simulink model "IEEE39BusSystem"  (R2024b)
settings: Solver=FixedStepDiscrete  StartTime=0.0  StopTime=15  FixedStep=Ts  MaxStep=1e-4  RelTol=1e-3
PreLoadFcn:
  | Ts = 1/60;
  | EnPSS = 1;
undefined symbols (not defined in the file): Gen1, Gen10, Gen2, Gen3, Gen4, Gen5, Gen6, Gen7, Gen8, Gen9, Load12, Load15, Load16, Load18, Load20, Load21, Load23, Load24, Load25, Load26, Load27, Load28, Load29, Load3, Load31, Load39, Load4, Load7, Load8
libraries: ee_lib x197, fl_lib x97, nesl_utility x91, eeGeneralControl x20, eeSmAC1C x10, eeSmPSS1A x10
(part 2 of 6)

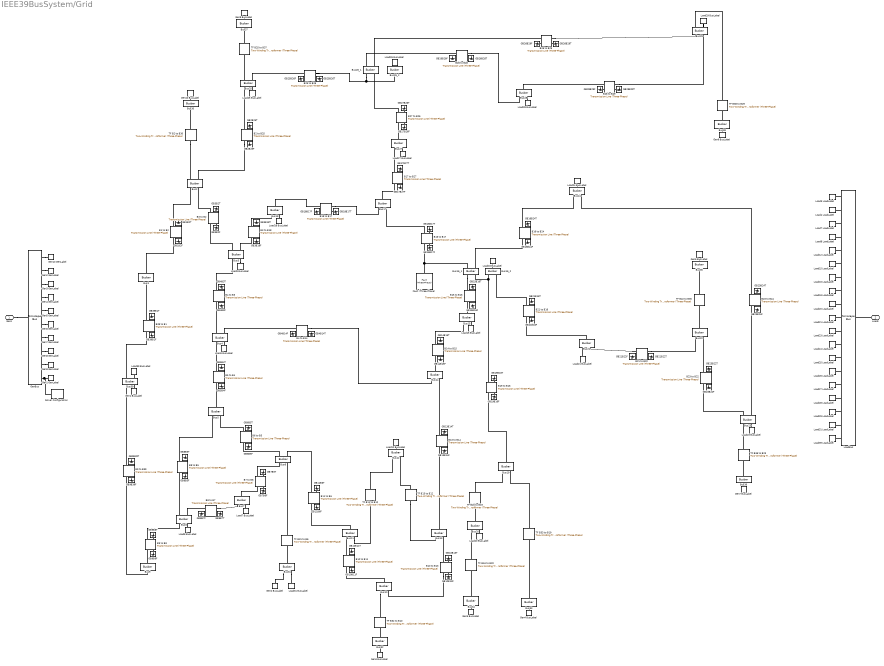
== system IEEE39BusSystem/Grid ==
  B1 to B2 : ee_lib/Passive/Lines/Transmission Line (Three-Phase)  length=1 km  freq=60 Hz  R=16.6635 Ohm/km  L=519.0496 mH/km  M=389.2872 mH/km  Cl=0.20762 uF/km  Cg=0.93427 uF/km  Rm=12.4976 Ohm/km  ModelTwoSections=ee.enum.enable.no  N=1  InterfacePosition=1 km  N1sec=1  N2sec=1  Access_ground=ee.enum.enable.no  R_parasitic=1e-6 Ohm  G_parasitic=1e-6 1/Ohm
      settings: InternalSimscapePortConfiguration="{\"Bottom\":[],\"Left\":[{\"id\":\"N1\",\"label\":\"~1\",\"type\":\"foundation.electrical.three_phase\"},{\"id\":\"g1\",\"label\":\"g1\",\"type\":\"foundation.electrical.electrical\"}],\"Right\":[{\"id\":\"N2\",\"label\":\"~2\",\"type\":\"foundation.electrical.three_phase\"},{\"id\":\"g2\",\"label\":\"g2\",\"type\":\"foundation.electrical.electrical\"}],\"Top\":[]}"
  B10 to B11 : ee_lib/Passive/Lines/Transmission Line (Three-Phase)  length=1 km  freq=60 Hz  R=1.9044 Ohm/km  L=54.3045 mH/km  M=40.7283 mH/km  Cl=0.021662 uF/km  Cg=0.097479 uF/km  Rm=1.4283 Ohm/km  ModelTwoSections=ee.enum.enable.no  N=1  InterfacePosition=1 km  N1sec=1  N2sec=1  Access_ground=ee.enum.enable.no  R_parasitic=1e-6 Ohm  G_parasitic=1e-6 1/Ohm
      settings: InternalSimscapePortConfiguration="{\"Bottom\":[],\"Left\":[{\"id\":\"N1\",\"label\":\"~1\",\"type\":\"foundation.electrical.three_phase\"},{\"id\":\"g1\",\"label\":\"g1\",\"type\":\"foundation.electrical.electrical\"}],\"Right\":[{\"id\":\"N2\",\"label\":\"~2\",\"type\":\"foundation.electrical.three_phase\"},{\"id\":\"g2\",\"label\":\"g2\",\"type\":\"foundation.electrical.electrical\"}],\"Top\":[]}"
  B10 to B13 : ee_lib/Passive/Lines/Transmission Line (Three-Phase)  length=1 km  freq=60 Hz  R=1.9044 Ohm/km  L=54.3045 mH/km  M=40.7283 mH/km  Cl=0.021662 uF/km  Cg=0.097479 uF/km  Rm=1.4283 Ohm/km  ModelTwoSections=ee.enum.enable.no  N=1  InterfacePosition=1 km  N1sec=1  N2sec=1  Access_ground=ee.enum.enable.no  R_parasitic=1e-6 Ohm  G_parasitic=1e-6 1/Ohm
      settings: InternalSimscapePortConfiguration="{\"Bottom\":[],\"Left\":[{\"id\":\"N1\",\"label\":\"~1\",\"type\":\"foundation.electrical.three_phase\"},{\"id\":\"g1\",\"label\":\"g1\",\"type\":\"foundation.electrical.electrical\"}],\"Right\":[{\"id\":\"N2\",\"label\":\"~2\",\"type\":\"foundation.electrical.three_phase\"},{\"id\":\"g2\",\"label\":\"g2\",\"type\":\"foundation.electrical.electrical\"}],\"Top\":[]}"
  B11 to B6 : ee_lib/Passive/Lines/Transmission Line (Three-Phase)  length=1 km  freq=60 Hz  R=3.3327 Ohm/km  L=103.5573 mH/km  M=77.668 mH/km  Cl=0.041274 uF/km  Cg=0.18573 uF/km  Rm=2.4995 Ohm/km  ModelTwoSections=ee.enum.enable.no  N=1  InterfacePosition=1 km  N1sec=1  N2sec=1  Access_ground=ee.enum.enable.no  R_parasitic=1e-6 Ohm  G_parasitic=1e-6 1/Ohm
      settings: InternalSimscapePortConfiguration="{\"Bottom\":[],\"Left\":[{\"id\":\"N1\",\"label\":\"~1\",\"type\":\"foundation.electrical.three_phase\"},{\"id\":\"g1\",\"label\":\"g1\",\"type\":\"foundation.electrical.electrical\"}],\"Right\":[{\"id\":\"N2\",\"label\":\"~2\",\"type\":\"foundation.electrical.three_phase\"},{\"id\":\"g2\",\"label\":\"g2\",\"type\":\"foundation.electrical.electrical\"}],\"Top\":[]}"
  B13 to B14 : ee_lib/Passive/Lines/Transmission Line (Three-Phase)  length=1 km  freq=60 Hz  R=4.2849 Ohm/km  L=127.5523 mH/km  M=95.6643 mH/km  Cl=0.051198 uF/km  Cg=0.23039 uF/km  Rm=3.2137 Ohm/km  ModelTwoSections=ee.enum.enable.no  N=1  InterfacePosition=1 km  N1sec=1  N2sec=1  Access_ground=ee.enum.enable.no  R_parasitic=1e-6 Ohm  G_parasitic=1e-6 1/Ohm
      settings: InternalSimscapePortConfiguration="{\"Bottom\":[],\"Left\":[{\"id\":\"N1\",\"label\":\"~1\",\"type\":\"foundation.electrical.three_phase\"},{\"id\":\"g1\",\"label\":\"g1\",\"type\":\"foundation.electrical.electrical\"}],\"Right\":[{\"id\":\"N2\",\"label\":\"~2\",\"type\":\"foundation.electrical.three_phase\"},{\"id\":\"g2\",\"label\":\"g2\",\"type\":\"foundation.electrical.electrical\"}],\"Top\":[]}"
  B14 to B15 : ee_lib/Passive/Lines/Transmission Line (Three-Phase)  length=1 km  freq=60 Hz  R=8.5698 Ohm/km  L=274.0481 mH/km  M=205.5361 mH/km  Cl=0.10876 uF/km  Cg=0.4894 uF/km  Rm=6.4273 Ohm/km  ModelTwoSections=ee.enum.enable.no  N=1  InterfacePosition=1 km  N1sec=1  N2sec=1  Access_ground=ee.enum.enable.no  R_parasitic=1e-6 Ohm  G_parasitic=1e-6 1/Ohm
      settings: InternalSimscapePortConfiguration="{\"Bottom\":[],\"Left\":[{\"id\":\"N1\",\"label\":\"~1\",\"type\":\"foundation.electrical.three_phase\"},{\"id\":\"g1\",\"label\":\"g1\",\"type\":\"foundation.electrical.electrical\"}],\"Right\":[{\"id\":\"N2\",\"label\":\"~2\",\"type\":\"foundation.electrical.three_phase\"},{\"id\":\"g2\",\"label\":\"g2\",\"type\":\"foundation.electrical.electrical\"}],\"Top\":[]}"
  B15 to B16 : ee_lib/Passive/Lines/Transmission Line (Three-Phase)  length=1 km  freq=60 Hz  R=4.2849 Ohm/km  L=118.7121 mH/km  M=89.0341 mH/km  Cl=0.050812 uF/km  Cg=0.22865 uF/km  Rm=3.2137 Ohm/km  ModelTwoSections=ee.enum.enable.no  N=1  InterfacePosition=1 km  N1sec=1  N2sec=1  Access_ground=ee.enum.enable.no  R_parasitic=1e-6 Ohm  G_parasitic=1e-6 1/Ohm
      settings: InternalSimscapePortConfiguration="{\"Bottom\":[],\"Left\":[{\"id\":\"N1\",\"label\":\"~1\",\"type\":\"foundation.electrical.three_phase\"},{\"id\":\"g1\",\"label\":\"g1\",\"type\":\"foundation.electrical.electrical\"}],\"Right\":[{\"id\":\"N2\",\"label\":\"~2\",\"type\":\"foundation.electrical.three_phase\"},{\"id\":\"g2\",\"label\":\"g2\",\"type\":\"foundation.electrical.electrical\"}],\"Top\":[]}"
  B16 to B17 : ee_lib/Passive/Lines/Transmission Line (Three-Phase)  length=1 km  freq=60 Hz  R=3.3327 Ohm/km  L=112.3976 mH/km  M=84.2982 mH/km  Cl=0.039877 uF/km  Cg=0.17945 uF/km  Rm=2.4995 Ohm/km  ModelTwoSections=ee.enum.enable.no  N=1  InterfacePosition=1 km  N1sec=1  N2sec=1  Access_ground=ee.enum.enable.no  R_parasitic=1e-6 Ohm  G_parasitic=1e-6 1/Ohm
      settings: InternalSimscapePortConfiguration="{\"Bottom\":[],\"Left\":[{\"id\":\"N1\",\"label\":\"~1\",\"type\":\"foundation.electrical.three_phase\"},{\"id\":\"g1\",\"label\":\"g1\",\"type\":\"foundation.electrical.electrical\"}],\"Right\":[{\"id\":\"N2\",\"label\":\"~2\",\"type\":\"foundation.electrical.three_phase\"},{\"id\":\"g2\",\"label\":\"g2\",\"type\":\"foundation.electrical.electrical\"}],\"Top\":[]}"
  B16 to B24 : ee_lib/Passive/Lines/Transmission Line (Three-Phase)  length=1 km  freq=60 Hz  R=1.4283 Ohm/km  L=74.5108 mH/km  M=55.8831 mH/km  Cl=0.020206 uF/km  Cg=0.090927 uF/km  Rm=1.0712 Ohm/km  ModelTwoSections=ee.enum.enable.no  N=1  InterfacePosition=1 km  N1sec=1  N2sec=1  Access_ground=ee.enum.enable.no  R_parasitic=1e-6 Ohm  G_parasitic=1e-6 1/Ohm
      settings: InternalSimscapePortConfiguration="{\"Bottom\":[],\"Left\":[{\"id\":\"N1\",\"label\":\"~1\",\"type\":\"foundation.electrical.three_phase\"},{\"id\":\"g1\",\"label\":\"g1\",\"type\":\"foundation.electrical.electrical\"}],\"Right\":[{\"id\":\"N2\",\"label\":\"~2\",\"type\":\"foundation.electrical.three_phase\"},{\"id\":\"g2\",\"label\":\"g2\",\"type\":\"foundation.electrical.electrical\"}],\"Top\":[]}"
  B17 to B27 : ee_lib/Passive/Lines/Transmission Line (Three-Phase)  length=1 km  freq=60 Hz  R=6.1893 Ohm/km  L=218.4807 mH/km  M=163.8606 mH/km  Cl=0.095562 uF/km  Cg=0.43003 uF/km  Rm=4.642 Ohm/km  ModelTwoSections=ee.enum.enable.no  N=1  InterfacePosition=1 km  N1sec=1  N2sec=1  Access_ground=ee.enum.enable.no  R_parasitic=1e-6 Ohm  G_parasitic=1e-6 1/Ohm
      settings: InternalSimscapePortConfiguration="{\"Bottom\":[],\"Left\":[{\"id\":\"N1\",\"label\":\"~1\",\"type\":\"foundation.electrical.three_phase\"},{\"id\":\"g1\",\"label\":\"g1\",\"type\":\"foundation.electrical.electrical\"}],\"Right\":[{\"id\":\"N2\",\"label\":\"~2\",\"type\":\"foundation.electrical.three_phase\"},{\"id\":\"g2\",\"label\":\"g2\",\"type\":\"foundation.electrical.electrical\"}],\"Top\":[]}"
  B18 to B17 : ee_lib/Passive/Lines/Transmission Line (Three-Phase)  length=1 km  freq=60 Hz  R=3.3327 Ohm/km  L=103.5573 mH/km  M=77.668 mH/km  Cl=0.039194 uF/km  Cg=0.17637 uF/km  Rm=2.4995 Ohm/km  ModelTwoSections=ee.enum.enable.no  N=1  InterfacePosition=1 km  N1sec=1  N2sec=1  Access_ground=ee.enum.enable.no  R_parasitic=1e-6 Ohm  G_parasitic=1e-6 1/Ohm
      settings: InternalSimscapePortConfiguration="{\"Bottom\":[],\"Left\":[{\"id\":\"N1\",\"label\":\"~1\",\"type\":\"foundation.electrical.three_phase\"},{\"id\":\"g1\",\"label\":\"g1\",\"type\":\"foundation.electrical.electrical\"}],\"Right\":[{\"id\":\"N2\",\"label\":\"~2\",\"type\":\"foundation.electrical.three_phase\"},{\"id\":\"g2\",\"label\":\"g2\",\"type\":\"foundation.electrical.electrical\"}],\"Top\":[]}"
  B19 to B16 : ee_lib/Passive/Lines/Transmission Line (Three-Phase)  length=1 km  freq=60 Hz  R=7.6176 Ohm/km  L=246.2644 mH/km  M=184.6983 mH/km  Cl=0.090332 uF/km  Cg=0.4065 uF/km  Rm=5.7132 Ohm/km  ModelTwoSections=ee.enum.enable.no  N=1  InterfacePosition=1 km  N1sec=1  N2sec=1  Access_ground=ee.enum.enable.no  R_parasitic=1e-6 Ohm  G_parasitic=1e-6 1/Ohm
      settings: InternalSimscapePortConfiguration="{\"Bottom\":[],\"Left\":[{\"id\":\"N1\",\"label\":\"~1\",\"type\":\"foundation.electrical.three_phase\"},{\"id\":\"g1\",\"label\":\"g1\",\"type\":\"foundation.electrical.electrical\"}],\"Right\":[{\"id\":\"N2\",\"label\":\"~2\",\"type\":\"foundation.electrical.three_phase\"},{\"id\":\"g2\",\"label\":\"g2\",\"type\":\"foundation.electrical.electrical\"}],\"Top\":[]}"
  B2 to B25 : ee_lib/Passive/Lines/Transmission Line (Three-Phase)  length=1 km  freq=60 Hz  R=33.327 Ohm/km  L=108.6089 mH/km  M=81.4567 mH/km  Cl=0.043383 uF/km  Cg=0.19522 uF/km  Rm=24.9952 Ohm/km  ModelTwoSections=ee.enum.enable.no  N=1  InterfacePosition=1 km  N1sec=1  N2sec=1  Access_ground=ee.enum.enable.no  R_parasitic=1e-6 Ohm  G_parasitic=1e-6 1/Ohm
      settings: InternalSimscapePortConfiguration="{\"Bottom\":[],\"Left\":[{\"id\":\"N1\",\"label\":\"~1\",\"type\":\"foundation.electrical.three_phase\"},{\"id\":\"g1\",\"label\":\"g1\",\"type\":\"foundation.electrical.electrical\"}],\"Right\":[{\"id\":\"N2\",\"label\":\"~2\",\"type\":\"foundation.electrical.three_phase\"},{\"id\":\"g2\",\"label\":\"g2\",\"type\":\"foundation.electrical.electrical\"}],\"Top\":[]}"
  B21 to B16 : ee_lib/Passive/Lines/Transmission Line (Three-Phase)  length=1 km  freq=60 Hz  R=3.8088 Ohm/km  L=170.4908 mH/km  M=127.8681 mH/km  Cl=0.075713 uF/km  Cg=0.34071 uF/km  Rm=2.8566 Ohm/km  ModelTwoSections=ee.enum.enable.no  N=1  InterfacePosition=1 km  N1sec=1  N2sec=1  Access_ground=ee.enum.enable.no  R_parasitic=1e-6 Ohm  G_parasitic=1e-6 1/Ohm
      settings: InternalSimscapePortConfiguration="{\"Bottom\":[],\"Left\":[{\"id\":\"N1\",\"label\":\"~1\",\"type\":\"foundation.electrical.three_phase\"},{\"id\":\"g1\",\"label\":\"g1\",\"type\":\"foundation.electrical.electrical\"}],\"Right\":[{\"id\":\"N2\",\"label\":\"~2\",\"type\":\"foundation.electrical.three_phase\"},{\"id\":\"g2\",\"label\":\"g2\",\"type\":\"foundation.electrical.electrical\"}],\"Top\":[]}"
  B21 to B22 : ee_lib/Passive/Lines/Transmission Line (Three-Phase)  length=1 km  freq=60 Hz  R=3.8088 Ohm/km  L=176.8052 mH/km  M=132.6039 mH/km  Cl=0.076218 uF/km  Cg=0.34298 uF/km  Rm=2.8566 Ohm/km  ModelTwoSections=ee.enum.enable.no  N=1  InterfacePosition=1 km  N1sec=1  N2sec=1  Access_ground=ee.enum.enable.no  R_parasitic=1e-6 Ohm  G_parasitic=1e-6 1/Ohm
      settings: InternalSimscapePortConfiguration="{\"Bottom\":[],\"Left\":[{\"id\":\"N1\",\"label\":\"~1\",\"type\":\"foundation.electrical.three_phase\"},{\"id\":\"g1\",\"label\":\"g1\",\"type\":\"foundation.electrical.electrical\"}],\"Right\":[{\"id\":\"N2\",\"label\":\"~2\",\"type\":\"foundation.electrical.three_phase\"},{\"id\":\"g2\",\"label\":\"g2\",\"type\":\"foundation.electrical.electrical\"}],\"Top\":[]}"
  B23 to B22 : ee_lib/Passive/Lines/Transmission Line (Three-Phase)  length=1 km  freq=60 Hz  R=2.8566 Ohm/km  L=121.2379 mH/km  M=90.9284 mH/km  Cl=0.054853 uF/km  Cg=0.24684 uF/km  Rm=2.1424 Ohm/km  ModelTwoSections=ee.enum.enable.no  N=1  InterfacePosition=1 km  N1sec=1  N2sec=1  Access_ground=ee.enum.enable.no  R_parasitic=1e-6 Ohm  G_parasitic=1e-6 1/Ohm
      settings: InternalSimscapePortConfiguration="{\"Bottom\":[],\"Left\":[{\"id\":\"N1\",\"label\":\"~1\",\"type\":\"foundation.electrical.three_phase\"},{\"id\":\"g1\",\"label\":\"g1\",\"type\":\"foundation.electrical.electrical\"}],\"Right\":[{\"id\":\"N2\",\"label\":\"~2\",\"type\":\"foundation.electrical.three_phase\"},{\"id\":\"g2\",\"label\":\"g2\",\"type\":\"foundation.electrical.electrical\"}],\"Top\":[]}"
  B23 to B24 : ee_lib/Passive/Lines/Transmission Line (Three-Phase)  length=1 km  freq=60 Hz  R=10.4742 Ohm/km  L=442.0131 mH/km  M=331.5098 mH/km  Cl=0.10727 uF/km  Cg=0.48271 uF/km  Rm=7.8557 Ohm/km  ModelTwoSections=ee.enum.enable.no  N=1  InterfacePosition=1 km  N1sec=1  N2sec=1  Access_ground=ee.enum.enable.no  R_parasitic=1e-6 Ohm  G_parasitic=1e-6 1/Ohm
      settings: InternalSimscapePortConfiguration="{\"Bottom\":[],\"Left\":[{\"id\":\"N1\",\"label\":\"~1\",\"type\":\"foundation.electrical.three_phase\"},{\"id\":\"g1\",\"label\":\"g1\",\"type\":\"foundation.electrical.electrical\"}],\"Right\":[{\"id\":\"N2\",\"label\":\"~2\",\"type\":\"foundation.electrical.three_phase\"},{\"id\":\"g2\",\"label\":\"g2\",\"type\":\"foundation.electrical.electrical\"}],\"Top\":[]}"
  B25 to B26 : ee_lib/Passive/Lines/Transmission Line (Three-Phase)  length=1 km  freq=60 Hz  R=15.2352 Ohm/km  L=407.9149 mH/km  M=305.9362 mH/km  Cl=0.15244 uF/km  Cg=0.68596 uF/km  Rm=11.4264 Ohm/km  ModelTwoSections=ee.enum.enable.no  N=1  InterfacePosition=1 km  N1sec=1  N2sec=1  Access_ground=ee.enum.enable.no  R_parasitic=1e-6 Ohm  G_parasitic=1e-6 1/Ohm
      settings: InternalSimscapePortConfiguration="{\"Bottom\":[],\"Left\":[{\"id\":\"N1\",\"label\":\"~1\",\"type\":\"foundation.electrical.three_phase\"},{\"id\":\"g1\",\"label\":\"g1\",\"type\":\"foundation.electrical.electrical\"}],\"Right\":[{\"id\":\"N2\",\"label\":\"~2\",\"type\":\"foundation.electrical.three_phase\"},{\"id\":\"g2\",\"label\":\"g2\",\"type\":\"foundation.electrical.electrical\"}],\"Top\":[]}"
  B26 to B28 : ee_lib/Passive/Lines/Transmission Line (Three-Phase)  length=1 km  freq=60 Hz  R=20.4723 Ohm/km  L=598.612 mH/km  M=448.959 mH/km  Cl=0.23183 uF/km  Cg=1.0432 uF/km  Rm=15.3542 Ohm/km  ModelTwoSections=ee.enum.enable.no  N=1  InterfacePosition=1 km  N1sec=1  N2sec=1  Access_ground=ee.enum.enable.no  R_parasitic=1e-6 Ohm  G_parasitic=1e-6 1/Ohm
      settings: InternalSimscapePortConfiguration="{\"Bottom\":[],\"Left\":[{\"id\":\"N1\",\"label\":\"~1\",\"type\":\"foundation.electrical.three_phase\"},{\"id\":\"g1\",\"label\":\"g1\",\"type\":\"foundation.electrical.electrical\"}],\"Right\":[{\"id\":\"N2\",\"label\":\"~2\",\"type\":\"foundation.electrical.three_phase\"},{\"id\":\"g2\",\"label\":\"g2\",\"type\":\"foundation.electrical.electrical\"}],\"Top\":[]}"
  B26 to B29 : ee_lib/Passive/Lines/Transmission Line (Three-Phase)  length=1 km  freq=60 Hz  R=27.1377 Ohm/km  L=789.309 mH/km  M=591.9818 mH/km  Cl=0.30576 uF/km  Cg=1.3759 uF/km  Rm=20.3533 Ohm/km  ModelTwoSections=ee.enum.enable.no  N=1  InterfacePosition=1 km  N1sec=1  N2sec=1  Access_ground=ee.enum.enable.no  R_parasitic=1e-6 Ohm  G_parasitic=1e-6 1/Ohm
      settings: InternalSimscapePortConfiguration="{\"Bottom\":[],\"Left\":[{\"id\":\"N1\",\"label\":\"~1\",\"type\":\"foundation.electrical.three_phase\"},{\"id\":\"g1\",\"label\":\"g1\",\"type\":\"foundation.electrical.electrical\"}],\"Right\":[{\"id\":\"N2\",\"label\":\"~2\",\"type\":\"foundation.electrical.three_phase\"},{\"id\":\"g2\",\"label\":\"g2\",\"type\":\"foundation.electrical.electrical\"}],\"Top\":[]}"
  B27 to B26 : ee_lib/Passive/Lines/Transmission Line (Three-Phase)  length=1 km  freq=60 Hz  R=6.6654 Ohm/km  L=185.6455 mH/km  M=139.2341 mH/km  Cl=0.071196 uF/km  Cg=0.32038 uF/km  Rm=4.999 Ohm/km  ModelTwoSections=ee.enum.enable.no  N=1  InterfacePosition=1 km  N1sec=1  N2sec=1  Access_ground=ee.enum.enable.no  R_parasitic=1e-6 Ohm  G_parasitic=1e-6 1/Ohm
      settings: InternalSimscapePortConfiguration="{\"Bottom\":[],\"Left\":[{\"id\":\"N1\",\"label\":\"~1\",\"type\":\"foundation.electrical.three_phase\"},{\"id\":\"g1\",\"label\":\"g1\",\"type\":\"foundation.electrical.electrical\"}],\"Right\":[{\"id\":\"N2\",\"label\":\"~2\",\"type\":\"foundation.electrical.three_phase\"},{\"id\":\"g2\",\"label\":\"g2\",\"type\":\"foundation.electrical.electrical\"}],\"Top\":[]}"
  B28 to B29 : ee_lib/Passive/Lines/Transmission Line (Three-Phase)  length=1 km  freq=60 Hz  R=6.6654 Ohm/km  L=190.6971 mH/km  M=143.0228 mH/km  Cl=0.073989 uF/km  Cg=0.33295 uF/km  Rm=4.999 Ohm/km  ModelTwoSections=ee.enum.enable.no  N=1  InterfacePosition=1 km  N1sec=1  N2sec=1  Access_ground=ee.enum.enable.no  R_parasitic=1e-6 Ohm  G_parasitic=1e-6 1/Ohm
      settings: InternalSimscapePortConfiguration="{\"Bottom\":[],\"Left\":[{\"id\":\"N1\",\"label\":\"~1\",\"type\":\"foundation.electrical.three_phase\"},{\"id\":\"g1\",\"label\":\"g1\",\"type\":\"foundation.electrical.electrical\"}],\"Right\":[{\"id\":\"N2\",\"label\":\"~2\",\"type\":\"foundation.electrical.three_phase\"},{\"id\":\"g2\",\"label\":\"g2\",\"type\":\"foundation.electrical.electrical\"}],\"Top\":[]}"
  B3 to B18 : ee_lib/Passive/Lines/Transmission Line (Three-Phase)  length=1 km  freq=60 Hz  R=5.2371 Ohm/km  L=167.965 mH/km  M=125.9737 mH/km  Cl=0.06353 uF/km  Cg=0.28588 uF/km  Rm=3.9278 Ohm/km  ModelTwoSections=ee.enum.enable.no  N=1  InterfacePosition=1 km  N1sec=1  N2sec=1  Access_ground=ee.enum.enable.no  R_parasitic=1e-6 Ohm  G_parasitic=1e-6 1/Ohm
      settings: InternalSimscapePortConfiguration="{\"Bottom\":[],\"Left\":[{\"id\":\"N1\",\"label\":\"~1\",\"type\":\"foundation.electrical.three_phase\"},{\"id\":\"g1\",\"label\":\"g1\",\"type\":\"foundation.electrical.electrical\"}],\"Right\":[{\"id\":\"N2\",\"label\":\"~2\",\"type\":\"foundation.electrical.three_phase\"},{\"id\":\"g2\",\"label\":\"g2\",\"type\":\"foundation.electrical.electrical\"}],\"Top\":[]}"
  B3 to B2 : ee_lib/Passive/Lines/Transmission Line (Three-Phase)  length=1 km  freq=60 Hz  R=6.1893 Ohm/km  L=190.6971 mH/km  M=143.0228 mH/km  Cl=0.076426 uF/km  Cg=0.34392 uF/km  Rm=4.642 Ohm/km  ModelTwoSections=ee.enum.enable.no  N=1  InterfacePosition=1 km  N1sec=1  N2sec=1  Access_ground=ee.enum.enable.no  R_parasitic=1e-6 Ohm  G_parasitic=1e-6 1/Ohm
      settings: InternalSimscapePortConfiguration="{\"Bottom\":[],\"Left\":[{\"id\":\"N1\",\"label\":\"~1\",\"type\":\"foundation.electrical.three_phase\"},{\"id\":\"g1\",\"label\":\"g1\",\"type\":\"foundation.electrical.electrical\"}],\"Right\":[{\"id\":\"N2\",\"label\":\"~2\",\"type\":\"foundation.electrical.three_phase\"},{\"id\":\"g2\",\"label\":\"g2\",\"type\":\"foundation.electrical.electrical\"}],\"Top\":[]}"
  B39 to B1 : ee_lib/Passive/Lines/Transmission Line (Three-Phase)  length=1 km  freq=60 Hz  R=4.761 Ohm/km  L=315.7236 mH/km  M=236.7927 mH/km  Cl=0.22286 uF/km  Cg=1.0029 uF/km  Rm=3.5707 Ohm/km  ModelTwoSections=ee.enum.enable.no  N=1  InterfacePosition=1 km  N1sec=1  N2sec=1  Access_ground=ee.enum.enable.no  R_parasitic=1e-6 Ohm  G_parasitic=1e-6 1/Ohm
      settings: InternalSimscapePortConfiguration="{\"Bottom\":[],\"Left\":[{\"id\":\"N1\",\"label\":\"~1\",\"type\":\"foundation.electrical.three_phase\"},{\"id\":\"g1\",\"label\":\"g1\",\"type\":\"foundation.electrical.electrical\"}],\"Right\":[{\"id\":\"N2\",\"label\":\"~2\",\"type\":\"foundation.electrical.three_phase\"},{\"id\":\"g2\",\"label\":\"g2\",\"type\":\"foundation.electrical.electrical\"}],\"Top\":[]}"
  B4 to B14 : ee_lib/Passive/Lines/Transmission Line (Three-Phase)  length=1 km  freq=60 Hz  R=3.8088 Ohm/km  L=162.9134 mH/km  M=122.185 mH/km  Cl=0.041066 uF/km  Cg=0.18479 uF/km  Rm=2.8566 Ohm/km  ModelTwoSections=ee.enum.enable.no  N=1  InterfacePosition=1 km  N1sec=1  N2sec=1  Access_ground=ee.enum.enable.no  R_parasitic=1e-6 Ohm  G_parasitic=1e-6 1/Ohm
      settings: InternalSimscapePortConfiguration="{\"Bottom\":[],\"Left\":[{\"id\":\"N1\",\"label\":\"~1\",\"type\":\"foundation.electrical.three_phase\"},{\"id\":\"g1\",\"label\":\"g1\",\"type\":\"foundation.electrical.electrical\"}],\"Right\":[{\"id\":\"N2\",\"label\":\"~2\",\"type\":\"foundation.electrical.three_phase\"},{\"id\":\"g2\",\"label\":\"g2\",\"type\":\"foundation.electrical.electrical\"}],\"Top\":[]}"
  B4 to B3 : ee_lib/Passive/Lines/Transmission Line (Three-Phase)  length=1 km  freq=60 Hz  R=6.1893 Ohm/km  L=268.9965 mH/km  M=201.7474 mH/km  Cl=0.065788 uF/km  Cg=0.29605 uF/km  Rm=4.642 Ohm/km  ModelTwoSections=ee.enum.enable.no  N=1  InterfacePosition=1 km  N1sec=1  N2sec=1  Access_ground=ee.enum.enable.no  R_parasitic=1e-6 Ohm  G_parasitic=1e-6 1/Ohm
      settings: InternalSimscapePortConfiguration="{\"Bottom\":[],\"Left\":[{\"id\":\"N1\",\"label\":\"~1\",\"type\":\"foundation.electrical.three_phase\"},{\"id\":\"g1\",\"label\":\"g1\",\"type\":\"foundation.electrical.electrical\"}],\"Right\":[{\"id\":\"N2\",\"label\":\"~2\",\"type\":\"foundation.electrical.three_phase\"},{\"id\":\"g2\",\"label\":\"g2\",\"type\":\"foundation.electrical.electrical\"}],\"Top\":[]}"
  B5 to B4 : ee_lib/Passive/Lines/Transmission Line (Three-Phase)  length=1 km  freq=60 Hz  R=3.8088 Ohm/km  L=162.9134 mH/km  M=122.185 mH/km  Cl=0.041066 uF/km  Cg=0.18479 uF/km  Rm=2.8566 Ohm/km  ModelTwoSections=ee.enum.enable.no  N=1  InterfacePosition=1 km  N1sec=1  N2sec=1  Access_ground=ee.enum.enable.no  R_parasitic=1e-6 Ohm  G_parasitic=1e-6 1/Ohm
      settings: InternalSimscapePortConfiguration="{\"Bottom\":[],\"Left\":[{\"id\":\"N1\",\"label\":\"~1\",\"type\":\"foundation.electrical.three_phase\"},{\"id\":\"g1\",\"label\":\"g1\",\"type\":\"foundation.electrical.electrical\"}],\"Right\":[{\"id\":\"N2\",\"label\":\"~2\",\"type\":\"foundation.electrical.three_phase\"},{\"id\":\"g2\",\"label\":\"g2\",\"type\":\"foundation.electrical.electrical\"}],\"Top\":[]}"
  B6 to B5 : ee_lib/Passive/Lines/Transmission Line (Three-Phase)  length=1 km  freq=60 Hz  R=0.9522 Ohm/km  L=32.8353 mH/km  M=24.6264 mH/km  Cl=0.012896 uF/km  Cg=0.058033 uF/km  Rm=0.71415 Ohm/km  ModelTwoSections=ee.enum.enable.no  N=1  InterfacePosition=1 km  N1sec=1  N2sec=1  Access_ground=ee.enum.enable.no  R_parasitic=1e-6 Ohm  G_parasitic=1e-6 1/Ohm
      settings: InternalSimscapePortConfiguration="{\"Bottom\":[],\"Left\":[{\"id\":\"N1\",\"label\":\"~1\",\"type\":\"foundation.electrical.three_phase\"},{\"id\":\"g1\",\"label\":\"g1\",\"type\":\"foundation.electrical.electrical\"}],\"Right\":[{\"id\":\"N2\",\"label\":\"~2\",\"type\":\"foundation.electrical.three_phase\"},{\"id\":\"g2\",\"label\":\"g2\",\"type\":\"foundation.electrical.electrical\"}],\"Top\":[]}"
  B7 to B6 : ee_lib/Passive/Lines/Transmission Line (Three-Phase)  length=1 km  freq=60 Hz  R=2.8566 Ohm/km  L=116.1863 mH/km  M=87.1397 mH/km  Cl=0.033577 uF/km  Cg=0.1511 uF/km  Rm=2.1424 Ohm/km  ModelTwoSections=ee.enum.enable.no  N=1  InterfacePosition=1 km  N1sec=1  N2sec=1  Access_ground=ee.enum.enable.no  R_parasitic=1e-6 Ohm  G_parasitic=1e-6 1/Ohm
      settings: InternalSimscapePortConfiguration="{\"Bottom\":[],\"Left\":[{\"id\":\"N1\",\"label\":\"~1\",\"type\":\"foundation.electrical.three_phase\"},{\"id\":\"g1\",\"label\":\"g1\",\"type\":\"foundation.electrical.electrical\"}],\"Right\":[{\"id\":\"N2\",\"label\":\"~2\",\"type\":\"foundation.electrical.three_phase\"},{\"id\":\"g2\",\"label\":\"g2\",\"type\":\"foundation.electrical.electrical\"}],\"Top\":[]}"
  B8 to B5 : ee_lib/Passive/Lines/Transmission Line (Three-Phase)  length=1 km  freq=60 Hz  R=3.8088 Ohm/km  L=141.4442 mH/km  M=106.0831 mH/km  Cl=0.043859 uF/km  Cg=0.19736 uF/km  Rm=2.8566 Ohm/km  ModelTwoSections=ee.enum.enable.no  N=1  InterfacePosition=1 km  N1sec=1  N2sec=1  Access_ground=ee.enum.enable.no  R_parasitic=1e-6 Ohm  G_parasitic=1e-6 1/Ohm
      settings: InternalSimscapePortConfiguration="{\"Bottom\":[],\"Left\":[{\"id\":\"N1\",\"label\":\"~1\",\"type\":\"foundation.electrical.three_phase\"},{\"id\":\"g1\",\"label\":\"g1\",\"type\":\"foundation.electrical.electrical\"}],\"Right\":[{\"id\":\"N2\",\"label\":\"~2\",\"type\":\"foundation.electrical.three_phase\"},{\"id\":\"g2\",\"label\":\"g2\",\"type\":\"foundation.electrical.electrical\"}],\"Top\":[]}"
  B8 to B7 : ee_lib/Passive/Lines/Transmission Line (Three-Phase)  length=1 km  freq=60 Hz  R=1.9044 Ohm/km  L=58.0931 mH/km  M=43.5699 mH/km  Cl=0.023177 uF/km  Cg=0.1043 uF/km  Rm=1.4283 Ohm/km  ModelTwoSections=ee.enum.enable.no  N=1  InterfacePosition=1 km  N1sec=1  N2sec=1  Access_ground=ee.enum.enable.no  R_parasitic=1e-6 Ohm  G_parasitic=1e-6 1/Ohm
      settings: InternalSimscapePortConfiguration="{\"Bottom\":[],\"Left\":[{\"id\":\"N1\",\"label\":\"~1\",\"type\":\"foundation.electrical.three_phase\"},{\"id\":\"g1\",\"label\":\"g1\",\"type\":\"foundation.electrical.electrical\"}],\"Right\":[{\"id\":\"N2\",\"label\":\"~2\",\"type\":\"foundation.electrical.three_phase\"},{\"id\":\"g2\",\"label\":\"g2\",\"type\":\"foundation.electrical.electrical\"}],\"Top\":[]}"
  B9 to B39 : ee_lib/Passive/Lines/Transmission Line (Three-Phase)  length=1 km  freq=60 Hz  R=4.761 Ohm/km  L=315.7236 mH/km  M=236.7927 mH/km  Cl=0.35657 uF/km  Cg=1.6046 uF/km  Rm=3.5707 Ohm/km  ModelTwoSections=ee.enum.enable.no  N=1  InterfacePosition=1 km  N1sec=1  N2sec=1  Access_ground=ee.enum.enable.no  R_parasitic=1e-6 Ohm  G_parasitic=1e-6 1/Ohm
      settings: InternalSimscapePortConfiguration="{\"Bottom\":[],\"Left\":[{\"id\":\"N1\",\"label\":\"~1\",\"type\":\"foundation.electrical.three_phase\"},{\"id\":\"g1\",\"label\":\"g1\",\"type\":\"foundation.electrical.electrical\"}],\"Right\":[{\"id\":\"N2\",\"label\":\"~2\",\"type\":\"foundation.electrical.three_phase\"},{\"id\":\"g2\",\"label\":\"g2\",\"type\":\"foundation.electrical.electrical\"}],\"Top\":[]}"
  B9 to B8 : ee_lib/Passive/Lines/Transmission Line (Three-Phase)  length=1 km  freq=60 Hz  R=10.9503 Ohm/km  L=458.4307 mH/km  M=343.823 mH/km  Cl=0.11303 uF/km  Cg=0.50865 uF/km  Rm=8.2127 Ohm/km  ModelTwoSections=ee.enum.enable.no  N=1  InterfacePosition=1 km  N1sec=1  N2sec=1  Access_ground=ee.enum.enable.no  R_parasitic=1e-6 Ohm  G_parasitic=1e-6 1/Ohm
      settings: InternalSimscapePortConfiguration="{\"Bottom\":[],\"Left\":[{\"id\":\"N1\",\"label\":\"~1\",\"type\":\"foundation.electrical.three_phase\"},{\"id\":\"g1\",\"label\":\"g1\",\"type\":\"foundation.electrical.electrical\"}],\"Right\":[{\"id\":\"N2\",\"label\":\"~2\",\"type\":\"foundation.electrical.three_phase\"},{\"id\":\"g2\",\"label\":\"g2\",\"type\":\"foundation.electrical.electrical\"}],\"Top\":[]}"
  Bus1 : ee_lib/Connectors & References/Busbar  Tag="1.036 pu\\n20.85 deg\\n-150.3  150.3 MW\\n19.1  -19.1 Mvar"  n_nodes=ee.enum.connectors.busbar_number_of_connections.two  VRated=345 kV  freq=60 Hz  show_ps=ee.enum.connectors.busbar_measurement.false
      settings: AttributesFormatString=%<Tag>  InternalSimscapePortConfiguration="{\"Bottom\":[],\"Left\":[{\"id\":\"N1\",\"label\":\"~1\",\"type\":\"foundation.electrical.three_phase\"}],\"Right\":[{\"id\":\"N2\",\"label\":\"~2\",\"type\":\"foundation.electrical.three_phase\"}],\"Top\":[]}"
  Bus10 : ee_lib/Connectors & References/Busbar  Tag="0.966 pu\\n25.54 deg\\n649.4 -366.4 -283.0 MW\\n36.0  -34.5   -1.5 Mvar"  n_nodes=ee.enum.connectors.busbar_number_of_connections.three  VRated=345 kV  freq=60 Hz  show_ps=ee.enum.connectors.busbar_measurement.false
      settings: AttributesFormatString=%<Tag>  InternalSimscapePortConfiguration="{\"Bottom\":[],\"Left\":[{\"id\":\"N1\",\"label\":\"~1\",\"type\":\"foundation.electrical.three_phase\"},{\"id\":\"N3\",\"label\":\"~3\",\"type\":\"foundation.electrical.three_phase\"}],\"Right\":[{\"id\":\"N2\",\"label\":\"~2\",\"type\":\"foundation.electrical.three_phase\"}],\"Top\":[]}"
  Bus11 : ee_lib/Connectors & References/Busbar  Tag="0.963 pu\\n24.57 deg\\n365.8 -365.8   -0.0 MW\\n35.0    3.5  -38.4 Mvar"  n_nodes=ee.enum.connectors.busbar_number_of_connections.three  VRated=345 kV  freq=60 Hz  show_ps=ee.enum.connectors.busbar_measurement.false
      settings: AttributesFormatString=%<Tag>  InternalSimscapePortConfiguration="{\"Bottom\":[],\"Left\":[{\"id\":\"N1\",\"label\":\"~1\",\"type\":\"foundation.electrical.three_phase\"},{\"id\":\"N3\",\"label\":\"~3\",\"type\":\"foundation.electrical.three_phase\"}],\"Right\":[{\"id\":\"N2\",\"label\":\"~2\",\"type\":\"foundation.electrical.three_phase\"}],\"Top\":[]}"
  Bus12 : ee_lib/Connectors & References/Busbar  Tag="0.945 pu\\n54.61 deg\\n-0.2   -7.6    7.8 MW\\n37.6  -78.6   41.1 Mvar"  n_nodes=ee.enum.connectors.busbar_number_of_connections.three  VRated=345 kV  freq=60 Hz  show_ps=ee.enum.connectors.busbar_measurement.false
      settings: AttributesFormatString=%<Tag>  InternalSimscapePortConfiguration="{\"Bottom\":[],\"Left\":[{\"id\":\"N1\",\"label\":\"~1\",\"type\":\"foundation.electrical.three_phase\"},{\"id\":\"N3\",\"label\":\"~3\",\"type\":\"foundation.electrical.three_phase\"}],\"Right\":[{\"id\":\"N2\",\"label\":\"~2\",\"type\":\"foundation.electrical.three_phase\"}],\"Top\":[]}"
  Bus13 : ee_lib/Connectors & References/Busbar  Tag="0.964 pu\\n24.79 deg\\n-8.0 -274.7  282.6 MW\\n-42.1   37.5    4.6 Mvar"  n_nodes=ee.enum.connectors.busbar_number_of_connections.three  VRated=345 kV  freq=60 Hz  show_ps=ee.enum.connectors.busbar_measurement.false
      settings: AttributesFormatString=%<Tag>  InternalSimscapePortConfiguration="{\"Bottom\":[],\"Left\":[{\"id\":\"N1\",\"label\":\"~1\",\"type\":\"foundation.electrical.three_phase\"},{\"id\":\"N3\",\"label\":\"~3\",\"type\":\"foundation.electrical.three_phase\"}],\"Right\":[{\"id\":\"N2\",\"label\":\"~2\",\"type\":\"foundation.electrical.three_phase\"}],\"Top\":[]}"
  Bus14 : ee_lib/Connectors & References/Busbar  Tag="0.965 pu\\n23.06 deg\\n-267.1   -6.8  273.9 MW\\n-19.3   49.0  -29.7 Mvar"  n_nodes=ee.enum.connectors.busbar_number_of_connections.three  VRated=345 kV  freq=60 Hz  show_ps=ee.enum.connectors.busbar_measurement.false
      settings: AttributesFormatString=%<Tag>  InternalSimscapePortConfiguration="{\"Bottom\":[],\"Left\":[{\"id\":\"N1\",\"label\":\"~1\",\"type\":\"foundation.electrical.three_phase\"},{\"id\":\"N3\",\"label\":\"~3\",\"type\":\"foundation.electrical.three_phase\"}],\"Right\":[{\"id\":\"N2\",\"label\":\"~2\",\"type\":\"foundation.electrical.three_phase\"}],\"Top\":[]}"
  Bus15 : ee_lib/Connectors & References/Busbar  Tag="0.972 pu\\n22.94 deg\\n6.8  295.8 -302.6 MW\\n-14.9  159.6 -144.7 Mvar"  n_nodes=ee.enum.connectors.busbar_number_of_connections.three  VRated=345 kV  freq=60 Hz  show_ps=ee.enum.connectors.busbar_measurement.false
      settings: AttributesFormatString=%<Tag>  InternalSimscapePortConfiguration="{\"Bottom\":[],\"Left\":[{\"id\":\"N1\",\"label\":\"~1\",\"type\":\"foundation.electrical.three_phase\"},{\"id\":\"N3\",\"label\":\"~3\",\"type\":\"foundation.electrical.three_phase\"}],\"Right\":[{\"id\":\"N2\",\"label\":\"~2\",\"type\":\"foundation.electrical.three_phase\"}],\"Top\":[]}"
  Bus16_1 : ee_lib/Connectors & References/Busbar  Tag="0.990 pu\\n24.51 deg\\n-296.9 -261.2  518.6   39.4 MW\\n-154.1   70.5  -52.7  136.3 Mvar"  n_nodes=ee.enum.connectors.busbar_number_of_connections.four  VRated=345 kV  freq=60 Hz  show_ps=ee.enum.connectors.busbar_measurement.false
      settings: AttributesFormatString=%<Tag>  InternalSimscapePortConfiguration="{\"Bottom\":[],\"Left\":[{\"id\":\"N1\",\"label\":\"~1\",\"type\":\"foundation.electrical.three_phase\"},{\"id\":\"N3\",\"label\":\"~3\",\"type\":\"foundation.electrical.three_phase\"}],\"Right\":[{\"id\":\"N2\",\"label\":\"~2\",\"type\":\"foundation.electrical.three_phase\"},{\"id\":\"N4\",\"label\":\"~4\",\"type\":\"foundation.electrical.three_phase\"}],\"Top\":[]}"
  Bus16_2 : ee_lib/Connectors & References/Busbar  Tag="0.990 pu\\n24.51 deg\\n-1.7 -322.6  324.3 MW\\n-0.2  -31.7   31.9 Mvar"  n_nodes=ee.enum.connectors.busbar_number_of_connections.three  VRated=345 kV  freq=60 Hz  show_ps=ee.enum.connectors.busbar_measurement.false
      settings: AttributesFormatString=%<Tag>  InternalSimscapePortConfiguration="{\"Bottom\":[],\"Left\":[{\"id\":\"N1\",\"label\":\"~1\",\"type\":\"foundation.electrical.three_phase\"},{\"id\":\"N3\",\"label\":\"~3\",\"type\":\"foundation.electrical.three_phase\"}],\"Right\":[{\"id\":\"N2\",\"label\":\"~2\",\"type\":\"foundation.electrical.three_phase\"}],\"Top\":[]}"
  Bus17 : ee_lib/Connectors & References/Busbar  Tag="0.994 pu\\n23.13 deg\\n-215.0  -45.6  260.6 MW\\n4.7   59.1  -63.9 Mvar"  n_nodes=ee.enum.connectors.busbar_number_of_connections.three  VRated=345 kV  freq=60 Hz  show_ps=ee.enum.connectors.busbar_measurement.false
      settings: AttributesFormatString=%<Tag>  InternalSimscapePortConfiguration="{\"Bottom\":[],\"Left\":[{\"id\":\"N1\",\"label\":\"~1\",\"type\":\"foundation.electrical.three_phase\"},{\"id\":\"N3\",\"label\":\"~3\",\"type\":\"foundation.electrical.three_phase\"}],\"Right\":[{\"id\":\"N2\",\"label\":\"~2\",\"type\":\"foundation.electrical.three_phase\"}],\"Top\":[]}"
  Bus18 : ee_lib/Connectors & References/Busbar  Tag="0.993 pu\\n22.11 deg\\n-58.9  214.7 -155.8 MW\\n25.1    4.5  -29.6 Mvar"  n_nodes=ee.enum.connectors.busbar_number_of_connections.three  VRated=345 kV  freq=60 Hz  show_ps=ee.enum.connectors.busbar_measurement.false
      settings: AttributesFormatString=%<Tag>  InternalSimscapePortConfiguration="{\"Bottom\":[],\"Left\":[{\"id\":\"N1\",\"label\":\"~1\",\"type\":\"foundation.electrical.three_phase\"},{\"id\":\"N3\",\"label\":\"~3\",\"type\":\"foundation.electrical.three_phase\"}],\"Right\":[{\"id\":\"N2\",\"label\":\"~2\",\"type\":\"foundation.electrical.three_phase\"}],\"Top\":[]}"
  Bus19 : ee_lib/Connectors & References/Busbar  Tag="0.991 pu\\n30.48 deg\\n-107.6 -521.4  629.0 MW\\n-15.6   28.7  -13.2 Mvar"  n_nodes=ee.enum.connectors.busbar_number_of_connections.three  VRated=345 kV  freq=60 Hz  show_ps=ee.enum.connectors.busbar_measurement.false
      settings: AttributesFormatString=%<Tag>  InternalSimscapePortConfiguration="{\"Bottom\":[],\"Left\":[{\"id\":\"N1\",\"label\":\"~1\",\"type\":\"foundation.electrical.three_phase\"},{\"id\":\"N3\",\"label\":\"~3\",\"type\":\"foundation.electrical.three_phase\"}],\"Right\":[{\"id\":\"N2\",\"label\":\"~2\",\"type\":\"foundation.electrical.three_phase\"}],\"Top\":[]}"
  Bus2 : ee_lib/Connectors & References/Busbar  Tag="1.020 pu\\n24.31 deg\\n-151.1  249.7 -325.3  226.7 MW\\n83.1  145.9 -143.0  -86.0 Mvar"  n_nodes=ee.enum.connectors.busbar_number_of_connections.four  VRated=345 kV  freq=60 Hz  show_ps=ee.enum.connectors.busbar_measurement.false
      settings: AttributesFormatString=%<Tag>  InternalSimscapePortConfiguration="{\"Bottom\":[],\"Left\":[{\"id\":\"N1\",\"label\":\"~1\",\"type\":\"foundation.electrical.three_phase\"},{\"id\":\"N3\",\"label\":\"~3\",\"type\":\"foundation.electrical.three_phase\"}],\"Right\":[{\"id\":\"N2\",\"label\":\"~2\",\"type\":\"foundation.electrical.three_phase\"},{\"id\":\"N4\",\"label\":\"~4\",\"type\":\"foundation.electrical.three_phase\"}],\"Top\":[]}"
  Bus20 : ee_lib/Connectors & References/Busbar  Tag="0.988 pu\\n29.61 deg\\n505.4  107.3 -612.7 MW\\n86.8   13.7 -100.5 Mvar"  n_nodes=ee.enum.connectors.busbar_number_of_connections.three  VRated=345 kV  freq=60 Hz  show_ps=ee.enum.connectors.busbar_measurement.false
      settings: AttributesFormatString=%<Tag>  InternalSimscapePortConfiguration="{\"Bottom\":[],\"Left\":[{\"id\":\"N1\",\"label\":\"~1\",\"type\":\"foundation.electrical.three_phase\"},{\"id\":\"N3\",\"label\":\"~3\",\"type\":\"foundation.electrical.three_phase\"}],\"Right\":[{\"id\":\"N2\",\"label\":\"~2\",\"type\":\"foundation.electrical.three_phase\"}],\"Top\":[]}"
  Bus21 : ee_lib/Connectors & References/Busbar  Tag="0.996 pu\\n27.05 deg\\n-272.0 -325.1  597.2 MW\\n-114.2  -21.3  135.5 Mvar"  n_nodes=ee.enum.connectors.busbar_number_of_connections.three  VRated=345 kV  freq=60 Hz  show_ps=ee.enum.connectors.busbar_measurement.false
      settings: AttributesFormatString=%<Tag>  InternalSimscapePortConfiguration="{\"Bottom\":[],\"Left\":[{\"id\":\"N1\",\"label\":\"~1\",\"type\":\"foundation.electrical.three_phase\"},{\"id\":\"N3\",\"label\":\"~3\",\"type\":\"foundation.electrical.three_phase\"}],\"Right\":[{\"id\":\"N2\",\"label\":\"~2\",\"type\":\"foundation.electrical.three_phase\"}],\"Top\":[]}"
  Bus22 : ee_lib/Connectors & References/Busbar  Tag="1.022 pu\\n31.70 deg\\n-600.2  649.4  -49.2 MW\\n-161.8  163.5   -1.8 Mvar"  n_nodes=ee.enum.connectors.busbar_number_of_connections.three  VRated=345 kV  freq=60 Hz  show_ps=ee.enum.connectors.busbar_measurement.false
      settings: AttributesFormatString=%<Tag>  InternalSimscapePortConfiguration="{\"Bottom\":[],\"Left\":[{\"id\":\"N1\",\"label\":\"~1\",\"type\":\"foundation.electrical.three_phase\"},{\"id\":\"N3\",\"label\":\"~3\",\"type\":\"foundation.electrical.three_phase\"}],\"Right\":[{\"id\":\"N2\",\"label\":\"~2\",\"type\":\"foundation.electrical.three_phase\"}],\"Top\":[]}"
  Bus23 : ee_lib/Connectors & References/Busbar  Tag="1.020 pu\\n31.45 deg\\n558.2   49.2 -257.7 -349.7 MW\\n112.0   20.8  -88.1  -44.7 Mvar"  n_nodes=ee.enum.connectors.busbar_number_of_connections.four  VRated=345 kV  freq=60 Hz  show_ps=ee.enum.connectors.busbar_measurement.false
      settings: AttributesFormatString=%<Tag>  InternalSimscapePortConfiguration="{\"Bottom\":[],\"Left\":[{\"id\":\"N1\",\"label\":\"~1\",\"type\":\"foundation.electrical.three_phase\"},{\"id\":\"N3\",\"label\":\"~3\",\"type\":\"foundation.electrical.three_phase\"}],\"Right\":[{\"id\":\"N2\",\"label\":\"~2\",\"type\":\"foundation.electrical.three_phase\"},{\"id\":\"N4\",\"label\":\"~4\",\"type\":\"foundation.electrical.three_phase\"}],\"Top\":[]}"
  Bus24 : ee_lib/Connectors & References/Busbar  Tag="0.998 pu\\n24.62 deg\\n-39.5 -307.5  347.0 MW\\n-130.7   91.7   39.1 Mvar"  n_nodes=ee.enum.connectors.busbar_number_of_connections.three  VRated=345 kV  freq=60 Hz  show_ps=ee.enum.connectors.busbar_measurement.false
      settings: AttributesFormatString=%<Tag>  InternalSimscapePortConfiguration="{\"Bottom\":[],\"Left\":[{\"id\":\"N1\",\"label\":\"~1\",\"type\":\"foundation.electrical.three_phase\"},{\"id\":\"N3\",\"label\":\"~3\",\"type\":\"foundation.electrical.three_phase\"}],\"Right\":[{\"id\":\"N2\",\"label\":\"~2\",\"type\":\"foundation.electrical.three_phase\"}],\"Top\":[]}"
  Bus25 : ee_lib/Connectors & References/Busbar  Tag="1.028 pu\\n25.73 deg\\n-230.7  538.1 -236.9  -70.5 MW\\n96.4  -48.7  -49.9    2.3 Mvar"  n_nodes=ee.enum.connectors.busbar_number_of_connections.four  VRated=345 kV  freq=60 Hz  show_ps=ee.enum.connectors.busbar_measurement.false
      settings: AttributesFormatString=%<Tag>  InternalSimscapePortConfiguration="{\"Bottom\":[],\"Left\":[{\"id\":\"N1\",\"label\":\"~1\",\"type\":\"foundation.electrical.three_phase\"},{\"id\":\"N3\",\"label\":\"~3\",\"type\":\"foundation.electrical.three_phase\"}],\"Right\":[{\"id\":\"N2\",\"label\":\"~2\",\"type\":\"foundation.electrical.three_phase\"},{\"id\":\"N4\",\"label\":\"~4\",\"type\":\"foundation.electrical.three_phase\"}],\"Top\":[]}"
  Bus26_1 : ee_lib/Connectors & References/Busbar  Tag="1.019 pu\\n24.53 deg\\n-73.9  129.9 -237.1  181.1 MW\\n32.1   26.2  -88.5   30.1 Mvar"  n_nodes=ee.enum.connectors.busbar_number_of_connections.four  VRated=345 kV  freq=60 Hz  show_ps=ee.enum.connectors.busbar_measurement.false
      settings: AttributesFormatString=%<Tag>  InternalSimscapePortConfiguration="{\"Bottom\":[],\"Left\":[{\"id\":\"N1\",\"label\":\"~1\",\"type\":\"foundation.electrical.three_phase\"},{\"id\":\"N3\",\"label\":\"~3\",\"type\":\"foundation.electrical.three_phase\"}],\"Right\":[{\"id\":\"N2\",\"label\":\"~2\",\"type\":\"foundation.electrical.three_phase\"},{\"id\":\"N4\",\"label\":\"~4\",\"type\":\"foundation.electrical.three_phase\"}],\"Top\":[]}"
  Bus26_2 : ee_lib/Connectors & References/Busbar  Tag="1.019 pu\\n24.53 deg\\n144.2 -144.2 MW\\n17.6  -17.6 Mvar"  n_nodes=ee.enum.connectors.busbar_number_of_connections.two  VRated=345 kV  freq=60 Hz  show_ps=ee.enum.connectors.busbar_measurement.false
      settings: AttributesFormatString=%<Tag>  InternalSimscapePortConfiguration="{\"Bottom\":[],\"Left\":[{\"id\":\"N1\",\"label\":\"~1\",\"type\":\"foundation.electrical.three_phase\"}],\"Right\":[{\"id\":\"N2\",\"label\":\"~2\",\"type\":\"foundation.electrical.three_phase\"}],\"Top\":[]}"
  Bus27 : ee_lib/Connectors & References/Busbar  Tag="1.001 pu\\n22.65 deg\\n45.5  236.2 -281.7 MW\\n-27.8  103.5  -75.7 Mvar"  n_nodes=ee.enum.connectors.busbar_number_of_connections.three  VRated=345 kV  freq=60 Hz  show_ps=ee.enum.connectors.busbar_measurement.false
      settings: AttributesFormatString=%<Tag>  InternalSimscapePortConfiguration="{\"Bottom\":[],\"Left\":[{\"id\":\"N1\",\"label\":\"~1\",\"type\":\"foundation.electrical.three_phase\"},{\"id\":\"N3\",\"label\":\"~3\",\"type\":\"foundation.electrical.three_phase\"}],\"Right\":[{\"id\":\"N2\",\"label\":\"~2\",\"type\":\"foundation.electrical.three_phase\"}],\"Top\":[]}"
  Bus28 : ee_lib/Connectors & References/Busbar  Tag="1.019 pu\\n27.96 deg\\n-130.6  344.6 -214.0 MW\\n47.0  -18.3  -28.7 Mvar"  n_nodes=ee.enum.connectors.busbar_number_of_connections.three  VRated=345 kV  freq=60 Hz  show_ps=ee.enum.connectors.busbar_measurement.false
      settings: AttributesFormatString=%<Tag>  InternalSimscapePortConfiguration="{\"Bottom\":[],\"Left\":[{\"id\":\"N1\",\"label\":\"~1\",\"type\":\"foundation.electrical.three_phase\"},{\"id\":\"N3\",\"label\":\"~3\",\"type\":\"foundation.electrical.three_phase\"}],\"Right\":[{\"id\":\"N2\",\"label\":\"~2\",\"type\":\"foundation.electrical.three_phase\"}],\"Top\":[]}"
  Bus29 : ee_lib/Connectors & References/Busbar  Tag="1.021 pu\\n30.85 deg\\n-183.0  824.5 -346.2 -295.4 MW\\n56.8  -55.6   26.8  -28.0 Mvar"  n_nodes=ee.enum.connectors.busbar_number_of_connections.four  VRated=345 kV  freq=60 Hz  show_ps=ee.enum.connectors.busbar_measurement.false
      settings: AttributesFormatString=%<Tag>  InternalSimscapePortConfiguration="{\"Bottom\":[],\"Left\":[{\"id\":\"N1\",\"label\":\"~1\",\"type\":\"foundation.electrical.three_phase\"},{\"id\":\"N3\",\"label\":\"~3\",\"type\":\"foundation.electrical.three_phase\"}],\"Right\":[{\"id\":\"N2\",\"label\":\"~2\",\"type\":\"foundation.electrical.three_phase\"},{\"id\":\"N4\",\"label\":\"~4\",\"type\":\"foundation.electrical.three_phase\"}],\"Top\":[]}"
  Bus3 : ee_lib/Connectors & References/Busbar  Tag="0.994 pu\\n21.65 deg\\n-64.2  323.6 -318.3   58.9 MW\\n-143.3  150.2   -2.4   -4.5 Mvar"  n_nodes=ee.enum.connectors.busbar_number_of_connections.four  VRated=345 kV  freq=60 Hz  show_ps=ee.enum.connectors.busbar_measurement.false
      settings: AttributesFormatString=%<Tag>  InternalSimscapePortConfiguration="{\"Bottom\":[],\"Left\":[{\"id\":\"N1\",\"label\":\"~1\",\"type\":\"foundation.electrical.three_phase\"},{\"id\":\"N3\",\"label\":\"~3\",\"type\":\"foundation.electrical.three_phase\"}],\"Right\":[{\"id\":\"N2\",\"label\":\"~2\",\"type\":\"foundation.electrical.three_phase\"},{\"id\":\"N4\",\"label\":\"~4\",\"type\":\"foundation.electrical.three_phase\"}],\"Top\":[]}"
  Bus30 : ee_lib/Connectors & References/Busbar  Tag="1.047 pu\\n-3.28 deg\\n-250.0  250.0 MW\\n-160.7  160.7 Mvar"  n_nodes=ee.enum.connectors.busbar_number_of_connections.two  VRated=22 kV  freq=60 Hz  show_ps=ee.enum.connectors.busbar_measurement.false
      settings: AttributesFormatString=%<Tag>  InternalSimscapePortConfiguration="{\"Bottom\":[],\"Left\":[{\"id\":\"N1\",\"label\":\"~1\",\"type\":\"foundation.electrical.three_phase\"}],\"Right\":[{\"id\":\"N2\",\"label\":\"~2\",\"type\":\"foundation.electrical.three_phase\"}],\"Top\":[]}"
  Bus31 : ee_lib/Connectors & References/Busbar  Tag="0.982 pu\\n0.00 deg\\n487.6 -478.8   -8.9 MW\\n118.5 -114.1   -4.4 Mvar"  n_nodes=ee.enum.connectors.busbar_number_of_connections.three  VRated=22 kV  freq=60 Hz  show_ps=ee.enum.connectors.busbar_measurement.false
      settings: AttributesFormatString=%<Tag>  InternalSimscapePortConfiguration="{\"Bottom\":[],\"Left\":[{\"id\":\"N1\",\"label\":\"~1\",\"type\":\"foundation.electrical.three_phase\"},{\"id\":\"N3\",\"label\":\"~3\",\"type\":\"foundation.electrical.three_phase\"}],\"Right\":[{\"id\":\"N2\",\"label\":\"~2\",\"type\":\"foundation.electrical.three_phase\"}],\"Top\":[]}"
  Bus32 : ee_lib/Connectors & References/Busbar  Tag=0.983 pu\n3.40 deg\n650.0 -650.0 MW\n126.9 -126.9 Mvar  n_nodes=ee.enum.connectors.busbar_number_of_connections.two  VRated=22 kV  freq=60 Hz  show_ps=ee.enum.connectors.busbar_measurement.false
      settings: AttributesFormatString=%<Tag>  InternalSimscapePortConfiguration="{\"Bottom\":[],\"Left\":[{\"id\":\"N1\",\"label\":\"~1\",\"type\":\"foundation.electrical.three_phase\"}],\"Right\":[{\"id\":\"N2\",\"label\":\"~2\",\"type\":\"foundation.electrical.three_phase\"}],\"Top\":[]}"
  Bus33 : ee_lib/Connectors & References/Busbar  Tag="0.997 pu\\n5.67 deg\\n632.0 -632.0 MW\\n44.3  -44.3 Mvar"  n_nodes=ee.enum.connectors.busbar_number_of_connections.two  VRated=22 kV  freq=60 Hz  show_ps=ee.enum.connectors.busbar_measurement.false
      settings: AttributesFormatString=%<Tag>  InternalSimscapePortConfiguration="{\"Bottom\":[],\"Left\":[{\"id\":\"N1\",\"label\":\"~1\",\"type\":\"foundation.electrical.three_phase\"}],\"Right\":[{\"id\":\"N2\",\"label\":\"~2\",\"type\":\"foundation.electrical.three_phase\"}],\"Top\":[]}"
  Bus34 : ee_lib/Connectors & References/Busbar  Tag=1.012 pu\n4.79 deg\n508.0 -508.0 MW\n135.5 -135.5 Mvar  n_nodes=ee.enum.connectors.busbar_number_of_connections.two  VRated=22 kV  freq=60 Hz  show_ps=ee.enum.connectors.busbar_measurement.false
      settings: AttributesFormatString=%<Tag>  InternalSimscapePortConfiguration="{\"Bottom\":[],\"Left\":[{\"id\":\"N1\",\"label\":\"~1\",\"type\":\"foundation.electrical.three_phase\"}],\"Right\":[{\"id\":\"N2\",\"label\":\"~2\",\"type\":\"foundation.electrical.three_phase\"}],\"Top\":[]}"
  Bus35 : ee_lib/Connectors & References/Busbar  Tag="1.049 pu\\n6.66 deg\\n-650.0  650.0 MW\\n-225.2  225.2 Mvar"  n_nodes=ee.enum.connectors.busbar_number_of_connections.two  VRated=22 kV  freq=60 Hz  show_ps=ee.enum.connectors.busbar_measurement.false
      settings: AttributesFormatString=%<Tag>  InternalSimscapePortConfiguration="{\"Bottom\":[],\"Left\":[{\"id\":\"N1\",\"label\":\"~1\",\"type\":\"foundation.electrical.three_phase\"}],\"Right\":[{\"id\":\"N2\",\"label\":\"~2\",\"type\":\"foundation.electrical.three_phase\"}],\"Top\":[]}"
  Bus36 : ee_lib/Connectors & References/Busbar  Tag=1.064 pu\n9.46 deg\n560.0 -560.0 MW\n197.0 -197.0 Mvar  n_nodes=ee.enum.connectors.busbar_number_of_connections.two  VRated=22 kV  freq=60 Hz  show_ps=ee.enum.connectors.busbar_measurement.false
      settings: AttributesFormatString=%<Tag>  InternalSimscapePortConfiguration="{\"Bottom\":[],\"Left\":[{\"id\":\"N1\",\"label\":\"~1\",\"type\":\"foundation.electrical.three_phase\"}],\"Right\":[{\"id\":\"N2\",\"label\":\"~2\",\"type\":\"foundation.electrical.three_phase\"}],\"Top\":[]}"
  Bus37 : ee_lib/Connectors & References/Busbar  Tag="1.028 pu\\n2.53 deg\\n-540.0  540.0 MW\\n-15.6   15.6 Mvar"  n_nodes=ee.enum.connectors.busbar_number_of_connections.two  VRated=22 kV  freq=60 Hz  show_ps=ee.enum.connectors.busbar_measurement.false
      settings: AttributesFormatString=%<Tag>  InternalSimscapePortConfiguration="{\"Bottom\":[],\"Left\":[{\"id\":\"N1\",\"label\":\"~1\",\"type\":\"foundation.electrical.three_phase\"}],\"Right\":[{\"id\":\"N2\",\"label\":\"~2\",\"type\":\"foundation.electrical.three_phase\"}],\"Top\":[]}"
  Bus38 : ee_lib/Connectors & References/Busbar  Tag="1.027 pu\\n7.93 deg\\n830.0 -830.0 MW\\n46.9  -46.9 Mvar"  n_nodes=ee.enum.connectors.busbar_number_of_connections.two  VRated=22 kV  freq=60 Hz  show_ps=ee.enum.connectors.busbar_measurement.false
      settings: AttributesFormatString=%<Tag>  InternalSimscapePortConfiguration="{\"Bottom\":[],\"Left\":[{\"id\":\"N1\",\"label\":\"~1\",\"type\":\"foundation.electrical.three_phase\"}],\"Right\":[{\"id\":\"N2\",\"label\":\"~2\",\"type\":\"foundation.electrical.three_phase\"}],\"Top\":[]}"
  Bus39 : ee_lib/Connectors & References/Busbar  Tag="1.030 pu\\n18.84 deg\\n21.2  150.1 1000.0-1171.2 MW\\n-16.4   55.6  226.0 -265.2 Mvar"  n_nodes=ee.enum.connectors.busbar_number_of_connections.four  VRated=345 kV  freq=60 Hz  show_ps=ee.enum.connectors.busbar_measurement.false
      settings: AttributesFormatString=%<Tag>  InternalSimscapePortConfiguration="{\"Bottom\":[],\"Left\":[{\"id\":\"N1\",\"label\":\"~1\",\"type\":\"foundation.electrical.three_phase\"},{\"id\":\"N3\",\"label\":\"~3\",\"type\":\"foundation.electrical.three_phase\"}],\"Right\":[{\"id\":\"N2\",\"label\":\"~2\",\"type\":\"foundation.electrical.three_phase\"},{\"id\":\"N4\",\"label\":\"~4\",\"type\":\"foundation.electrical.three_phase\"}],\"Top\":[]}"
  Bus4 : ee_lib/Connectors & References/Busbar  Tag="0.960 pu\\n20.95 deg\\n130.8   63.9 -461.2  266.5 MW\\n-10.9  158.5 -169.7   22.1 Mvar"  n_nodes=ee.enum.connectors.busbar_number_of_connections.four  VRated=345 kV  freq=60 Hz  show_ps=ee.enum.connectors.busbar_measurement.false
      settings: AttributesFormatString=%<Tag>  InternalSimscapePortConfiguration="{\"Bottom\":[],\"Left\":[{\"id\":\"N1\",\"label\":\"~1\",\"type\":\"foundation.electrical.three_phase\"},{\"id\":\"N3\",\"label\":\"~3\",\"type\":\"foundation.electrical.three_phase\"}],\"Right\":[{\"id\":\"N2\",\"label\":\"~2\",\"type\":\"foundation.electrical.three_phase\"},{\"id\":\"N4\",\"label\":\"~4\",\"type\":\"foundation.electrical.three_phase\"}],\"Top\":[]}"
  Bus5 : ee_lib/Connectors & References/Busbar  Tag="0.959 pu\\n22.01 deg\\n-308.4 -130.9  439.4 MW\\n-20.8   21.2   -0.4 Mvar"  n_nodes=ee.enum.connectors.busbar_number_of_connections.three  VRated=345 kV  freq=60 Hz  show_ps=ee.enum.connectors.busbar_measurement.false
      settings: AttributesFormatString=%<Tag>  InternalSimscapePortConfiguration="{\"Bottom\":[],\"Left\":[{\"id\":\"N1\",\"label\":\"~1\",\"type\":\"foundation.electrical.three_phase\"},{\"id\":\"N3\",\"label\":\"~3\",\"type\":\"foundation.electrical.three_phase\"}],\"Right\":[{\"id\":\"N2\",\"label\":\"~2\",\"type\":\"foundation.electrical.three_phase\"}],\"Top\":[]}"
  Bus6 : ee_lib/Connectors & References/Busbar  Tag="0.960 pu\\n22.72 deg\\n-403.3 -439.8  478.3  364.7 MW\\n-47.6   -1.1   51.1   -2.5 Mvar"  n_nodes=ee.enum.connectors.busbar_number_of_connections.four  VRated=345 kV  freq=60 Hz  show_ps=ee.enum.connectors.busbar_measurement.false
      settings: AttributesFormatString=%<Tag>  InternalSimscapePortConfiguration="{\"Bottom\":[],\"Left\":[{\"id\":\"N1\",\"label\":\"~1\",\"type\":\"foundation.electrical.three_phase\"},{\"id\":\"N3\",\"label\":\"~3\",\"type\":\"foundation.electrical.three_phase\"}],\"Right\":[{\"id\":\"N2\",\"label\":\"~2\",\"type\":\"foundation.electrical.three_phase\"},{\"id\":\"N4\",\"label\":\"~4\",\"type\":\"foundation.electrical.three_phase\"}],\"Top\":[]}"
  Bus7 : ee_lib/Connectors & References/Busbar  Tag="0.953 pu\\n20.41 deg\\n-189.7  402.2 -212.5 MW\\n34.9   41.4  -76.4 Mvar"  n_nodes=ee.enum.connectors.busbar_number_of_connections.three  VRated=345 kV  freq=60 Hz  show_ps=ee.enum.connectors.busbar_measurement.false
      settings: AttributesFormatString=%<Tag>  InternalSimscapePortConfiguration="{\"Bottom\":[],\"Left\":[{\"id\":\"N1\",\"label\":\"~1\",\"type\":\"foundation.electrical.three_phase\"},{\"id\":\"N3\",\"label\":\"~3\",\"type\":\"foundation.electrical.three_phase\"}],\"Right\":[{\"id\":\"N2\",\"label\":\"~2\",\"type\":\"foundation.electrical.three_phase\"}],\"Top\":[]}"
  Bus8 : ee_lib/Connectors & References/Busbar  Tag="0.954 pu\\n19.86 deg\\n-21.8  307.6 -475.3  189.5 MW\\n167.3   22.6 -160.2  -29.7 Mvar"  n_nodes=ee.enum.connectors.busbar_number_of_connections.four  VRated=345 kV  freq=60 Hz  show_ps=ee.enum.connectors.busbar_measurement.false
      settings: AttributesFormatString=%<Tag>  InternalSimscapePortConfiguration="{\"Bottom\":[],\"Left\":[{\"id\":\"N1\",\"label\":\"~1\",\"type\":\"foundation.electrical.three_phase\"},{\"id\":\"N3\",\"label\":\"~3\",\"type\":\"foundation.electrical.three_phase\"}],\"Right\":[{\"id\":\"N2\",\"label\":\"~2\",\"type\":\"foundation.electrical.three_phase\"},{\"id\":\"N4\",\"label\":\"~4\",\"type\":\"foundation.electrical.three_phase\"}],\"Top\":[]}"
  Bus9 : ee_lib/Connectors & References/Busbar  Tag="1.011 pu\\n19.18 deg\\n-21.2   21.2 MW\\n139.7 -139.7 Mvar"  n_nodes=ee.enum.connectors.busbar_number_of_connections.two  VRated=345 kV  freq=60 Hz  show_ps=ee.enum.connectors.busbar_measurement.false
      settings: AttributesFormatString=%<Tag>  InternalSimscapePortConfiguration="{\"Bottom\":[],\"Left\":[{\"id\":\"N1\",\"label\":\"~1\",\"type\":\"foundation.electrical.three_phase\"}],\"Right\":[{\"id\":\"N2\",\"label\":\"~2\",\"type\":\"foundation.electrical.three_phase\"}],\"Top\":[]}"
  Fault (Three-Phase) : ee_lib/Utilities/Fault (Three-Phase)  fault_type_option=11  R_pn_fault=1e-3 Ohm  R_ng_fault=1e-3 Ohm  exposemeasurement=ee.enum.exposemeasurement.hidden  enable_external_fault=ee.enum.external_fault.hidden  fault_threshold=0.5  fault_condition=1  fault_resettable=0  enable_temporal_fault=1  fault_start_time=5 s  fault_duration=0.1 s  G_parasitic=1e-6 1/Ohm
      settings: InternalSimscapePortConfiguration="{\"Bottom\":[],\"Left\":[{\"id\":\"N\",\"label\":\"~\",\"type\":\"foundation.electrical.three_phase\"}],\"Right\":[],\"Top\":[]}"
  GB10B11F : fl_lib/Electrical/Electrical Elements/Electrical Reference
  GB10B11T : fl_lib/Electrical/Electrical Elements/Electrical Reference
  GB10B13F : fl_lib/Electrical/Electrical Elements/Electrical Reference
  GB10B13T : fl_lib/Electrical/Electrical Elements/Electrical Reference
  GB11B6F : fl_lib/Electrical/Electrical Elements/Electrical Reference
  GB11B6T : fl_lib/Electrical/Electrical Elements/Electrical Reference
  GB13B14F : fl_lib/Electrical/Electrical Elements/Electrical Reference
  GB13B14T : fl_lib/Electrical/Electrical Elements/Electrical Reference
  GB14B15F : fl_lib/Electrical/Electrical Elements/Electrical Reference
  GB14B15T : fl_lib/Electrical/Electrical Elements/Electrical Reference
  GB15B16F : fl_lib/Electrical/Electrical Elements/Electrical Reference
  GB15B16T : fl_lib/Electrical/Electrical Elements/Electrical Reference
  GB16B17F : fl_lib/Electrical/Electrical Elements/Electrical Reference
  GB16B17T : fl_lib/Electrical/Electrical Elements/Electrical Reference
  GB16B24F : fl_lib/Electrical/Electrical Elements/Electrical Reference
  GB16B24T : fl_lib/Electrical/Electrical Elements/Electrical Reference
  GB17B27F : fl_lib/Electrical/Electrical Elements/Electrical Reference
  GB17B27T : fl_lib/Electrical/Electrical Elements/Electrical Reference
  GB18B17F : fl_lib/Electrical/Electrical Elements/Electrical Reference
  GB18B17T : fl_lib/Electrical/Electrical Elements/Electrical Reference
  GB19B16F : fl_lib/Electrical/Electrical Elements/Electrical Reference
  GB19B16T : fl_lib/Electrical/Electrical Elements/Electrical Reference
  GB1B2F : fl_lib/Electrical/Electrical Elements/Electrical Reference
  GB1B2T : fl_lib/Electrical/Electrical Elements/Electrical Reference
  GB21B16F : fl_lib/Electrical/Electrical Elements/Electrical Reference
  GB21B16T : fl_lib/Electrical/Electrical Elements/Electrical Reference
  GB21B22F : fl_lib/Electrical/Electrical Elements/Electrical Reference
  GB21B22T : fl_lib/Electrical/Electrical Elements/Electrical Reference
  GB23B22F : fl_lib/Electrical/Electrical Elements/Electrical Reference
  GB23B22T : fl_lib/Electrical/Electrical Elements/Electrical Reference
  GB23B24F : fl_lib/Electrical/Electrical Elements/Electrical Reference
  GB23B24T : fl_lib/Electrical/Electrical Elements/Electrical Reference
  GB25B26F : fl_lib/Electrical/Electrical Elements/Electrical Reference
  GB25B26T : fl_lib/Electrical/Electrical Elements/Electrical Reference
  GB26B28F : fl_lib/Electrical/Electrical Elements/Electrical Reference
  GB26B28T : fl_lib/Electrical/Electrical Elements/Electrical Reference
  GB26B29F : fl_lib/Electrical/Electrical Elements/Electrical Reference
  GB26B29T : fl_lib/Electrical/Electrical Elements/Electrical Reference
  GB27B26F : fl_lib/Electrical/Electrical Elements/Electrical Reference
  GB27B26T : fl_lib/Electrical/Electrical Elements/Electrical Reference
  GB28B29F : fl_lib/Electrical/Electrical Elements/Electrical Reference
  GB28B29T : fl_lib/Electrical/Electrical Elements/Electrical Reference
  GB2B25F : fl_lib/Electrical/Electrical Elements/Electrical Reference
  GB2B25T : fl_lib/Electrical/Electrical Elements/Electrical Reference
  GB39B1F : fl_lib/Electrical/Electrical Elements/Electrical Reference
  GB39B1T : fl_lib/Electrical/Electrical Elements/Electrical Reference
  GB3B18F : fl_lib/Electrical/Electrical Elements/Electrical Reference
  GB3B18T : fl_lib/Electrical/Electrical Elements/Electrical Reference
  GB3B2F : fl_lib/Electrical/Electrical Elements/Electrical Reference
  GB3B2T : fl_lib/Electrical/Electrical Elements/Electrical Reference
  GB4B14F : fl_lib/Electrical/Electrical Elements/Electrical Reference
  GB4B14T : fl_lib/Electrical/Electrical Elements/Electrical Reference
  GB4B3F : fl_lib/Electrical/Electrical Elements/Electrical Reference
  GB4B3T : fl_lib/Electrical/Electrical Elements/Electrical Reference
  GB5B4F : fl_lib/Electrical/Electrical Elements/Electrical Reference
  GB5B4T : fl_lib/Electrical/Electrical Elements/Electrical Reference
  GB6B5F : fl_lib/Electrical/Electrical Elements/Electrical Reference
  GB6B5T : fl_lib/Electrical/Electrical Elements/Electrical Reference
  GB7B6F : fl_lib/Electrical/Electrical Elements/Electrical Reference
  GB7B6T : fl_lib/Electrical/Electrical Elements/Electrical Reference
  GB8B5F : fl_lib/Electrical/Electrical Elements/Electrical Reference
  GB8B5T : fl_lib/Electrical/Electrical Elements/Electrical Reference
  GB8B7F : fl_lib/Electrical/Electrical Elements/Electrical Reference
  GB8B7T : fl_lib/Electrical/Electrical Elements/Electrical Reference
  GB9B39F : fl_lib/Electrical/Electrical Elements/Electrical Reference
  GB9B39T : fl_lib/Electrical/Electrical Elements/Electrical Reference
  GB9B8F : fl_lib/Electrical/Electrical Elements/Electrical Reference
  GB9B8T : fl_lib/Electrical/Electrical Elements/Electrical Reference
  Gen1 BusLabel : ConnectionLabel  Label=Gen1Label
  Gen1 GenLabel : ConnectionLabel  Label=Gen1Label
  Gen10 BusLabel : ConnectionLabel  Label=Gen10Label
  Gen10 GenLabel : ConnectionLabel  Label=Gen10Label
  Gen2 BusLabel : ConnectionLabel  Label=Gen2Label
  Gen2 GenLabel : ConnectionLabel  Label=Gen2Label
  Gen3 BusLabel : ConnectionLabel  Label=Gen3Label
  Gen3 GenLabel : ConnectionLabel  Label=Gen3Label
  Gen4 BusLabel : ConnectionLabel  Label=Gen4Label
  Gen4 GenLabel : ConnectionLabel  Label=Gen4Label
  Gen5 BusLabel : ConnectionLabel  Label=Gen5Label
  Gen5 GenLabel : ConnectionLabel  Label=Gen5Label
  Gen6 BusLabel : ConnectionLabel  Label=Gen6Label
  Gen6 GenLabel : ConnectionLabel  Label=Gen6Label
  Gen7 BusLabel : ConnectionLabel  Label=Gen7Label
  Gen7 GenLabel : ConnectionLabel  Label=Gen7Label
  Gen8 BusLabel : ConnectionLabel  Label=Gen8Label
  Gen8 GenLabel : ConnectionLabel  Label=Gen8Label
  Gen9 BusLabel : ConnectionLabel  Label=Gen9Label
  Gen9 GenLabel : ConnectionLabel  Label=Gen9Label
  GenBus : SimscapeBus  HierarchyStrings=Gen10;Gen2;Gen3;Gen4;Gen5;Gen6;Gen7;Gen8;Gen9;Gen1
  Load12 BusLabel : ConnectionLabel  Label=Load12Label
  Load12 LoadLabel : ConnectionLabel  Label=Load12Label
  Load15 BusLabel : ConnectionLabel  Label=Load15Label
  Load15 LoadLabel : ConnectionLabel  Label=Load15Label
  Load16 BusLabel : ConnectionLabel  Label=Load16Label
  Load16 LoadLabel : ConnectionLabel  Label=Load16Label
  Load18 BusLabel : ConnectionLabel  Label=Load18Label
  Load18 LoadLabel : ConnectionLabel  Label=Load18Label
  Load20 BusLabel : ConnectionLabel  Label=Load20Label
  Load20 LoadLabel : ConnectionLabel  Label=Load20Label
  Load21 BusLabel : ConnectionLabel  Label=Load21Label
  Load21 LoadLabel : ConnectionLabel  Label=Load21Label
  Load23 BusLabel : ConnectionLabel  Label=Load23Label
  Load23 LoadLabel : ConnectionLabel  Label=Load23Label
  Load24 BusLabel : ConnectionLabel  Label=Load24Label
  Load24 LoadLabel : ConnectionLabel  Label=Load24Label
  Load25 BusLabel : ConnectionLabel  Label=Load25Label
  Load25 LoadLabel : ConnectionLabel  Label=Load25Label
  Load26 BusLabel : ConnectionLabel  Label=Load26Label
  Load26 LoadLabel : ConnectionLabel  Label=Load26Label
  Load27 BusLabel : ConnectionLabel  Label=Load27Label
  Load27 LoadLabel : ConnectionLabel  Label=Load27Label
  Load28 BusLabel : ConnectionLabel  Label=Load28Label
  Load28 LoadLabel : ConnectionLabel  Label=Load28Label
  Load29 BusLabel : ConnectionLabel  Label=Load29Label
  Load29 LoadLabel : ConnectionLabel  Label=Load29Label
  Load3 BusLabel : ConnectionLabel  Label=Load3Label
  Load3 LoadLabel : ConnectionLabel  Label=Load3Label
  Load31 BusLabel : ConnectionLabel  Label=Load31Label
  Load31 LoadLabel : ConnectionLabel  Label=Load31Label
  Load39 BusLabel : ConnectionLabel  Label=Load39Label
  Load39 LoadLabel : ConnectionLabel  Label=Load39Label
  Load4 BusLabel : ConnectionLabel  Label=Load4Label
  Load4 LoadLabel : ConnectionLabel  Label=Load4Label
  Load7 BusLabel : ConnectionLabel  Label=Load7Label
  Load7 LoadLabel : ConnectionLabel  Label=Load7Label
  Load8 BusLabel : ConnectionLabel  Label=Load8Label
  Load8 LoadLabel : ConnectionLabel  Label=Load8Label
  LoadBus : SimscapeBus  HierarchyStrings=Load3;Load4;Load7;Load8;Load12;Load15;Load16;Load18;Load20;Load21;Load23;Load24;Load25;Load26;Load27;Load28;Load29;Load31;Load39
  Solver Configuration : nesl_utility/Solver Configuration  PhysicalDomain=network_engine_domain  SubClassName=solver  LeftPortType=input  RightPortType=generic  Tones=[]  Harmonics=[]  SimulateNoise=off  Profile=off  UseLocalSampling=off  EnableSwitchedLinearOptims=on  FrequencyDomain=off  UseCCode=off  RelTol=0.001  AbsTol=0.001  MinStep=1e-09  ToWorkspace=off  RevertToSquareIcSolve=off  NumHomotopyIterations=100  PhasorMode=off  PhasorModeNumHarmonics=1  ConsistencySolver=NEWTON_FTOL  IndexReductionMethod=DerivativeReplacement  DoDC=off  ResidualTolerance=1e-09  ConsistencyTolSource=GLOBAL  ConsistencyAbsTol=0.001  ConsistencyRelTol=0.001  ConsistencyTolFactor=0.001  UseLocalSolver=on  LocalSolverChoice=NE_BACKWARD_EULER_ADVANCER  ResolveIndetEquations=on  FunctionEvalNumThread=1  LocalSolverSampleTime=Ts  DoFixedCost=on  MaxNonlinIter=3  MaxModeIter=2  ComputeImpulses=off  ImpulseIterations=2  LinearAlgebra=auto  LinearAlgebraNumThread=0  EquationFormulation=NE_FREQUENCY_TIME_EF  DelaysMemoryBudget=1024  AutomaticFiltering=on  FilteringTimeConstant=0.001  PartitionStorageMethod=AS_NEEDED  PartitionMemoryBudget=1024  PartitionMethod=ROBUST  MultibodyUseLocalSolver=off  MultibodyLocalSolverChoice=ODE1  MultibodyLocalSolverSampleTime=0.001
  TF B11 to B12 : ee_lib/Passive/Transformers/Two-Winding Transformer (Three-Phase)  SRated=100 MW  FRated=60 Hz  Winding1Connection=ee.enum.windingconnection.delta1  VRated1=345 kV  Winding2Connection=ee.enum.windingconnection.Yg  VRated2=345 kV  CoreType=ee.enum.coretype.fivelimb  pu_Rw1=0.0008  pu_Rw2=0.0008  leakage_reactance_option=ee.enum.transformer_leakage.include  pu_Xl1=0.02175  pu_Xl2=0.02175  magnetizing_resistance_option=ee.enum.transformer_magnetizingResistance.include  pu_Rm=500  magnetizing_reactance_option=ee.enum.transformer_magnetizingReactance.include  saturation_option=ee.enum.transformer_saturation.exclude  pu_Xm=500  current_data=[0, .002, 1, 2]  magnetic_flux_data=[0, 1.2, 1.5, 1.51]  pu_X0=0.5  i1_specify=off  i1_priority=None  i1=[0, 0, 0] A  i1_nominal_specify=off  i1_nominal_value=1  i1_nominal_unit=A  i2_specify=off  i2_priority=None  i2=[0, 0, 0] A  i2_nominal_specify=off  i2_nominal_value=1  i2_nominal_unit=A  phi_specify=off  phi_priority=None  phi=[0, 0, 0]  phi_nominal_specify=off  phi_nominal_value=1  phi_nominal_unit=1  power_dissipated_specify=off  power_dissipated_priority=None  power_dissipated=0 W  power_dissipated_nominal_specify=off  power_dissipated_nominal_value=1  power_dissipated_nominal_unit=W
      settings: InternalSimscapePortConfiguration="{\"Bottom\":[],\"Left\":[{\"id\":\"N1\",\"label\":\"~1\",\"type\":\"foundation.electrical.three_phase\"}],\"Right\":[{\"id\":\"N2\",\"label\":\"~2\",\"type\":\"foundation.electrical.three_phase\"}],\"Top\":[]}"
  TF B13 to B12 : ee_lib/Passive/Transformers/Two-Winding Transformer (Three-Phase)  SRated=100 MW  FRated=60 Hz  Winding1Connection=ee.enum.windingconnection.delta1  VRated1=345 kV  Winding2Connection=ee.enum.windingconnection.Yg  VRated2=345 kV  CoreType=ee.enum.coretype.fivelimb  pu_Rw1=0.0008  pu_Rw2=0.0008  leakage_reactance_option=ee.enum.transformer_leakage.include  pu_Xl1=0.02175  pu_Xl2=0.02175  magnetizing_resistance_option=ee.enum.transformer_magnetizingResistance.include  pu_Rm=500  magnetizing_reactance_option=ee.enum.transformer_magnetizingReactance.include  saturation_option=ee.enum.transformer_saturation.exclude  pu_Xm=500  current_data=[0, .002, 1, 2]  magnetic_flux_data=[0, 1.2, 1.5, 1.51]  pu_X0=0.5  i1_specify=off  i1_priority=None  i1=[0, 0, 0] A  i1_nominal_specify=off  i1_nominal_value=1  i1_nominal_unit=A  i2_specify=off  i2_priority=None  i2=[0, 0, 0] A  i2_nominal_specify=off  i2_nominal_value=1  i2_nominal_unit=A  phi_specify=off  phi_priority=None  phi=[0, 0, 0]  phi_nominal_specify=off  phi_nominal_value=1  phi_nominal_unit=1  power_dissipated_specify=off  power_dissipated_priority=None  power_dissipated=0 W  power_dissipated_nominal_specify=off  power_dissipated_nominal_value=1  power_dissipated_nominal_unit=W
      settings: InternalSimscapePortConfiguration="{\"Bottom\":[],\"Left\":[{\"id\":\"N1\",\"label\":\"~1\",\"type\":\"foundation.electrical.three_phase\"}],\"Right\":[{\"id\":\"N2\",\"label\":\"~2\",\"type\":\"foundation.electrical.three_phase\"}],\"Top\":[]}"
  TF B2 to B30 : ee_lib/Passive/Transformers/Two-Winding Transformer (Three-Phase)  SRated=100 MW  FRated=60 Hz  Winding1Connection=ee.enum.windingconnection.Yg  VRated1=345 kV  Winding2Connection=ee.enum.windingconnection.delta1  VRated2=22 kV  CoreType=ee.enum.coretype.fivelimb  pu_Rw1=5e-05  pu_Rw2=5e-05  leakage_reactance_option=ee.enum.transformer_leakage.include  pu_Xl1=0.00905  pu_Xl2=0.00905  magnetizing_resistance_option=ee.enum.transformer_magnetizingResistance.include  pu_Rm=500  magnetizing_reactance_option=ee.enum.transformer_magnetizingReactance.include  saturation_option=ee.enum.transformer_saturation.exclude  pu_Xm=500  current_data=[0, .002, 1, 2]  magnetic_flux_data=[0, 1.2, 1.5, 1.51]  pu_X0=0.5  i1_specify=off  i1_priority=None  i1=[0, 0, 0] A  i1_nominal_specify=off  i1_nominal_value=1  i1_nominal_unit=A  i2_specify=off  i2_priority=None  i2=[0, 0, 0] A  i2_nominal_specify=off  i2_nominal_value=1  i2_nominal_unit=A  phi_specify=off  phi_priority=None  phi=[0, 0, 0]  phi_nominal_specify=off  phi_nominal_value=1  phi_nominal_unit=1  power_dissipated_specify=off  power_dissipated_priority=None  power_dissipated=0 W  power_dissipated_nominal_specify=off  power_dissipated_nominal_value=1  power_dissipated_nominal_unit=W
      settings: InternalSimscapePortConfiguration="{\"Bottom\":[],\"Left\":[{\"id\":\"N1\",\"label\":\"~1\",\"type\":\"foundation.electrical.three_phase\"}],\"Right\":[{\"id\":\"N2\",\"label\":\"~2\",\"type\":\"foundation.electrical.three_phase\"}],\"Top\":[]}"
  TF B20 to B19 : ee_lib/Passive/Transformers/Two-Winding Transformer (Three-Phase)  SRated=100 MW  FRated=60 Hz  Winding1Connection=ee.enum.windingconnection.delta1  VRated1=345 kV  Winding2Connection=ee.enum.windingconnection.delta1  VRated2=345 kV  CoreType=ee.enum.coretype.fivelimb  pu_Rw1=0.00035  pu_Rw2=0.00035  leakage_reactance_option=ee.enum.transformer_leakage.include  pu_Xl1=0.0069  pu_Xl2=0.0069  magnetizing_resistance_option=ee.enum.transformer_magnetizingResistance.include  pu_Rm=500  magnetizing_reactance_option=ee.enum.transformer_magnetizingReactance.include  saturation_option=ee.enum.transformer_saturation.exclude  pu_Xm=500  current_data=[0, .002, 1, 2]  magnetic_flux_data=[0, 1.2, 1.5, 1.51]  pu_X0=0.5  i1_specify=off  i1_priority=None  i1=[0, 0, 0] A  i1_nominal_specify=off  i1_nominal_value=1  i1_nominal_unit=A  i2_specify=off  i2_priority=None  i2=[0, 0, 0] A  i2_nominal_specify=off  i2_nominal_value=1  i2_nominal_unit=A  phi_specify=off  phi_priority=None  phi=[0, 0, 0]  phi_nominal_specify=off  phi_nominal_value=1  phi_nominal_unit=1  power_dissipated_specify=off  power_dissipated_priority=None  power_dissipated=0 W  power_dissipated_nominal_specify=off  power_dissipated_nominal_value=1  power_dissipated_nominal_unit=W
      settings: InternalSimscapePortConfiguration="{\"Bottom\":[],\"Left\":[{\"id\":\"N1\",\"label\":\"~1\",\"type\":\"foundation.electrical.three_phase\"}],\"Right\":[{\"id\":\"N2\",\"label\":\"~2\",\"type\":\"foundation.electrical.three_phase\"}],\"Top\":[]}"
  TF B22 to B35 : ee_lib/Passive/Transformers/Two-Winding Transformer (Three-Phase)  SRated=100 MW  FRated=60 Hz  Winding1Connection=ee.enum.windingconnection.Yg  VRated1=345 kV  Winding2Connection=ee.enum.windingconnection.delta1  VRated2=22 kV  CoreType=ee.enum.coretype.fivelimb  pu_Rw1=5e-05  pu_Rw2=5e-05  leakage_reactance_option=ee.enum.transformer_leakage.include  pu_Xl1=0.00715  pu_Xl2=0.00715  magnetizing_resistance_option=ee.enum.transformer_magnetizingResistance.include  pu_Rm=500  magnetizing_reactance_option=ee.enum.transformer_magnetizingReactance.include  saturation_option=ee.enum.transformer_saturation.exclude  pu_Xm=500  current_data=[0, .002, 1, 2]  magnetic_flux_data=[0, 1.2, 1.5, 1.51]  pu_X0=0.5  i1_specify=off  i1_priority=None  i1=[0, 0, 0] A  i1_nominal_specify=off  i1_nominal_value=1  i1_nominal_unit=A  i2_specify=off  i2_priority=None  i2=[0, 0, 0] A  i2_nominal_specify=off  i2_nominal_value=1  i2_nominal_unit=A  phi_specify=off  phi_priority=None  phi=[0, 0, 0]  phi_nominal_specify=off  phi_nominal_value=1  phi_nominal_unit=1  power_dissipated_specify=off  power_dissipated_priority=None  power_dissipated=0 W  power_dissipated_nominal_specify=off  power_dissipated_nominal_value=1  power_dissipated_nominal_unit=W
      settings: InternalSimscapePortConfiguration="{\"Bottom\":[],\"Left\":[{\"id\":\"N1\",\"label\":\"~1\",\"type\":\"foundation.electrical.three_phase\"}],\"Right\":[{\"id\":\"N2\",\"label\":\"~2\",\"type\":\"foundation.electrical.three_phase\"}],\"Top\":[]}"
  TF B25 to B37 : ee_lib/Passive/Transformers/Two-Winding Transformer (Three-Phase)  SRated=100 MW  FRated=60 Hz  Winding1Connection=ee.enum.windingconnection.Yg  VRated1=345 kV  Winding2Connection=ee.enum.windingconnection.delta1  VRated2=22 kV  CoreType=ee.enum.coretype.fivelimb  pu_Rw1=0.0003  pu_Rw2=0.0003  leakage_reactance_option=ee.enum.transformer_leakage.include  pu_Xl1=0.0116  pu_Xl2=0.0116  magnetizing_resistance_option=ee.enum.transformer_magnetizingResistance.include  pu_Rm=500  magnetizing_reactance_option=ee.enum.transformer_magnetizingReactance.include  saturation_option=ee.enum.transformer_saturation.exclude  pu_Xm=500  current_data=[0, .002, 1, 2]  magnetic_flux_data=[0, 1.2, 1.5, 1.51]  pu_X0=0.5  i1_specify=off  i1_priority=None  i1=[0, 0, 0] A  i1_nominal_specify=off  i1_nominal_value=1  i1_nominal_unit=A  i2_specify=off  i2_priority=None  i2=[0, 0, 0] A  i2_nominal_specify=off  i2_nominal_value=1  i2_nominal_unit=A  phi_specify=off  phi_priority=None  phi=[0, 0, 0]  phi_nominal_specify=off  phi_nominal_value=1  phi_nominal_unit=1  power_dissipated_specify=off  power_dissipated_priority=None  power_dissipated=0 W  power_dissipated_nominal_specify=off  power_dissipated_nominal_value=1  power_dissipated_nominal_unit=W
      settings: InternalSimscapePortConfiguration="{\"Bottom\":[],\"Left\":[{\"id\":\"N1\",\"label\":\"~1\",\"type\":\"foundation.electrical.three_phase\"}],\"Right\":[{\"id\":\"N2\",\"label\":\"~2\",\"type\":\"foundation.electrical.three_phase\"}],\"Top\":[]}"
  TF B31 to B6 : ee_lib/Passive/Transformers/Two-Winding Transformer (Three-Phase)  SRated=100 MW  FRated=60 Hz  Winding1Connection=ee.enum.windingconnection.delta1  VRated1=22 kV  Winding2Connection=ee.enum.windingconnection.Yg  VRated2=345 kV  CoreType=ee.enum.coretype.fivelimb  pu_Rw1=5e-05  pu_Rw2=5e-05  leakage_reactance_option=ee.enum.transformer_leakage.include  pu_Xl1=0.0125  pu_Xl2=0.0125  magnetizing_resistance_option=ee.enum.transformer_magnetizingResistance.include  pu_Rm=500  magnetizing_reactance_option=ee.enum.transformer_magnetizingReactance.include  saturation_option=ee.enum.transformer_saturation.exclude  pu_Xm=500  current_data=[0, .002, 1, 2]  magnetic_flux_data=[0, 1.2, 1.5, 1.51]  pu_X0=0.5  i1_specify=off  i1_priority=None  i1=[0, 0, 0] A  i1_nominal_specify=off  i1_nominal_value=1  i1_nominal_unit=A  i2_specify=off  i2_priority=None  i2=[0, 0, 0] A  i2_nominal_specify=off  i2_nominal_value=1  i2_nominal_unit=A  phi_specify=off  phi_priority=None  phi=[0, 0, 0]  phi_nominal_specify=off  phi_nominal_value=1  phi_nominal_unit=1  power_dissipated_specify=off  power_dissipated_priority=None  power_dissipated=0 W  power_dissipated_nominal_specify=off  power_dissipated_nominal_value=1  power_dissipated_nominal_unit=W
      settings: InternalSimscapePortConfiguration="{\"Bottom\":[],\"Left\":[{\"id\":\"N1\",\"label\":\"~1\",\"type\":\"foundation.electrical.three_phase\"}],\"Right\":[{\"id\":\"N2\",\"label\":\"~2\",\"type\":\"foundation.electrical.three_phase\"}],\"Top\":[]}"
  TF B32 to B10 : ee_lib/Passive/Transformers/Two-Winding Transformer (Three-Phase)  SRated=100 MW  FRated=60 Hz  Winding1Connection=ee.enum.windingconnection.delta1  VRated1=22 kV  Winding2Connection=ee.enum.windingconnection.Yg  VRated2=345 kV  CoreType=ee.enum.coretype.fivelimb  pu_Rw1=5e-05  pu_Rw2=5e-05  leakage_reactance_option=ee.enum.transformer_leakage.include  pu_Xl1=0.01  pu_Xl2=0.01  magnetizing_resistance_option=ee.enum.transformer_magnetizingResistance.include  pu_Rm=500  magnetizing_reactance_option=ee.enum.transformer_magnetizingReactance.include  saturation_option=ee.enum.transformer_saturation.exclude  pu_Xm=500  current_data=[0, .002, 1, 2]  magnetic_flux_data=[0, 1.2, 1.5, 1.51]  pu_X0=0.5  i1_specify=off  i1_priority=None  i1=[0, 0, 0] A  i1_nominal_specify=off  i1_nominal_value=1  i1_nominal_unit=A  i2_specify=off  i2_priority=None  i2=[0, 0, 0] A  i2_nominal_specify=off  i2_nominal_value=1  i2_nominal_unit=A  phi_specify=off  phi_priority=None  phi=[0, 0, 0]  phi_nominal_specify=off  phi_nominal_value=1  phi_nominal_unit=1  power_dissipated_specify=off  power_dissipated_priority=None  power_dissipated=0 W  power_dissipated_nominal_specify=off  power_dissipated_nominal_value=1  power_dissipated_nominal_unit=W
      settings: InternalSimscapePortConfiguration="{\"Bottom\":[],\"Left\":[{\"id\":\"N1\",\"label\":\"~1\",\"type\":\"foundation.electrical.three_phase\"}],\"Right\":[{\"id\":\"N2\",\"label\":\"~2\",\"type\":\"foundation.electrical.three_phase\"}],\"Top\":[]}"
  TF B33 to B19 : ee_lib/Passive/Transformers/Two-Winding Transformer (Three-Phase)  SRated=100 MW  FRated=60 Hz  Winding1Connection=ee.enum.windingconnection.delta1  VRated1=22 kV  Winding2Connection=ee.enum.windingconnection.Yg  VRated2=345 kV  CoreType=ee.enum.coretype.fivelimb  pu_Rw1=0.00035  pu_Rw2=0.00035  leakage_reactance_option=ee.enum.transformer_leakage.include  pu_Xl1=0.0071  pu_Xl2=0.0071  magnetizing_resistance_option=ee.enum.transformer_magnetizingResistance.include  pu_Rm=500  magnetizing_reactance_option=ee.enum.transformer_magnetizingReactance.include  saturation_option=ee.enum.transformer_saturation.exclude  pu_Xm=500  current_data=[0, .002, 1, 2]  magnetic_flux_data=[0, 1.2, 1.5, 1.51]  pu_X0=0.5  i1_specify=off  i1_priority=None  i1=[0, 0, 0] A  i1_nominal_specify=off  i1_nominal_value=1  i1_nominal_unit=A  i2_specify=off  i2_priority=None  i2=[0, 0, 0] A  i2_nominal_specify=off  i2_nominal_value=1  i2_nominal_unit=A  phi_specify=off  phi_priority=None  phi=[0, 0, 0]  phi_nominal_specify=off  phi_nominal_value=1  phi_nominal_unit=1  power_dissipated_specify=off  power_dissipated_priority=None  power_dissipated=0 W  power_dissipated_nominal_specify=off  power_dissipated_nominal_value=1  power_dissipated_nominal_unit=W
      settings: InternalSimscapePortConfiguration="{\"Bottom\":[],\"Left\":[{\"id\":\"N1\",\"label\":\"~1\",\"type\":\"foundation.electrical.three_phase\"}],\"Right\":[{\"id\":\"N2\",\"label\":\"~2\",\"type\":\"foundation.electrical.three_phase\"}],\"Top\":[]}"
  TF B34 to B20 : ee_lib/Passive/Transformers/Two-Winding Transformer (Three-Phase)  SRated=100 MW  FRated=60 Hz  Winding1Connection=ee.enum.windingconnection.delta1  VRated1=22 kV  Winding2Connection=ee.enum.windingconnection.Yg  VRated2=345 kV  CoreType=ee.enum.coretype.fivelimb  pu_Rw1=0.00045  pu_Rw2=0.00045  leakage_reactance_option=ee.enum.transformer_leakage.include  pu_Xl1=0.009  pu_Xl2=0.009  magnetizing_resistance_option=ee.enum.transformer_magnetizingResistance.include  pu_Rm=500  magnetizing_reactance_option=ee.enum.transformer_magnetizingReactance.include  saturation_option=ee.enum.transformer_saturation.exclude  pu_Xm=500  current_data=[0, .002, 1, 2]  magnetic_flux_data=[0, 1.2, 1.5, 1.51]  pu_X0=0.5  i1_specify=off  i1_priority=None  i1=[0, 0, 0] A  i1_nominal_specify=off  i1_nominal_value=1  i1_nominal_unit=A  i2_specify=off  i2_priority=None  i2=[0, 0, 0] A  i2_nominal_specify=off  i2_nominal_value=1  i2_nominal_unit=A  phi_specify=off  phi_priority=None  phi=[0, 0, 0]  phi_nominal_specify=off  phi_nominal_value=1  phi_nominal_unit=1  power_dissipated_specify=off  power_dissipated_priority=None  power_dissipated=0 W  power_dissipated_nominal_specify=off  power_dissipated_nominal_value=1  power_dissipated_nominal_unit=W
      settings: InternalSimscapePortConfiguration="{\"Bottom\":[],\"Left\":[{\"id\":\"N1\",\"label\":\"~1\",\"type\":\"foundation.electrical.three_phase\"}],\"Right\":[{\"id\":\"N2\",\"label\":\"~2\",\"type\":\"foundation.electrical.three_phase\"}],\"Top\":[]}"
  TF B36 to B23 : ee_lib/Passive/Transformers/Two-Winding Transformer (Three-Phase)  SRated=100 MW  FRated=60 Hz  Winding1Connection=ee.enum.windingconnection.delta1  VRated1=22 kV  Winding2Connection=ee.enum.windingconnection.Yg  VRated2=345 kV  CoreType=ee.enum.coretype.fivelimb  pu_Rw1=0.00025  pu_Rw2=0.00025  leakage_reactance_option=ee.enum.transformer_leakage.include  pu_Xl1=0.0136  pu_Xl2=0.0136  magnetizing_resistance_option=ee.enum.transformer_magnetizingResistance.include  pu_Rm=500  magnetizing_reactance_option=ee.enum.transformer_magnetizingReactance.include  saturation_option=ee.enum.transformer_saturation.exclude  pu_Xm=500  current_data=[0, .002, 1, 2]  magnetic_flux_data=[0, 1.2, 1.5, 1.51]  pu_X0=0.5  i1_specify=off  i1_priority=None  i1=[0, 0, 0] A  i1_nominal_specify=off  i1_nominal_value=1  i1_nominal_unit=A  i2_specify=off  i2_priority=None  i2=[0, 0, 0] A  i2_nominal_specify=off  i2_nominal_value=1  i2_nominal_unit=A  phi_specify=off  phi_priority=None  phi=[0, 0, 0]  phi_nominal_specify=off  phi_nominal_value=1  phi_nominal_unit=1  power_dissipated_specify=off  power_dissipated_priority=None  power_dissipated=0 W  power_dissipated_nominal_specify=off  power_dissipated_nominal_value=1  power_dissipated_nominal_unit=W
      settings: InternalSimscapePortConfiguration="{\"Bottom\":[],\"Left\":[{\"id\":\"N1\",\"label\":\"~1\",\"type\":\"foundation.electrical.three_phase\"}],\"Right\":[{\"id\":\"N2\",\"label\":\"~2\",\"type\":\"foundation.electrical.three_phase\"}],\"Top\":[]}"
  TF B38 to B29 : ee_lib/Passive/Transformers/Two-Winding Transformer (Three-Phase)  SRated=100 MW  FRated=60 Hz  Winding1Connection=ee.enum.windingconnection.delta1  VRated1=22 kV  Winding2Connection=ee.enum.windingconnection.Yg  VRated2=345 kV  CoreType=ee.enum.coretype.fivelimb  pu_Rw1=0.0004  pu_Rw2=0.0004  leakage_reactance_option=ee.enum.transformer_leakage.include  pu_Xl1=0.0078  pu_Xl2=0.0078  magnetizing_resistance_option=ee.enum.transformer_magnetizingResistance.include  pu_Rm=500  magnetizing_reactance_option=ee.enum.transformer_magnetizingReactance.include  saturation_option=ee.enum.transformer_saturation.exclude  pu_Xm=500  current_data=[0, .002, 1, 2]  magnetic_flux_data=[0, 1.2, 1.5, 1.51]  pu_X0=0.5  i1_specify=off  i1_priority=None  i1=[0, 0, 0] A  i1_nominal_specify=off  i1_nominal_value=1  i1_nominal_unit=A  i2_specify=off  i2_priority=None  i2=[0, 0, 0] A  i2_nominal_specify=off  i2_nominal_value=1  i2_nominal_unit=A  phi_specify=off  phi_priority=None  phi=[0, 0, 0]  phi_nominal_specify=off  phi_nominal_value=1  phi_nominal_unit=1  power_dissipated_specify=off  power_dissipated_priority=None  power_dissipated=0 W  power_dissipated_nominal_specify=off  power_dissipated_nominal_value=1  power_dissipated_nominal_unit=W
      settings: InternalSimscapePortConfiguration="{\"Bottom\":[],\"Left\":[{\"id\":\"N1\",\"label\":\"~1\",\"type\":\"foundation.electrical.three_phase\"}],\"Right\":[{\"id\":\"N2\",\"label\":\"~2\",\"type\":\"foundation.electrical.three_phase\"}],\"Top\":[]}"
  Gens : PMIOPort  Side=Left
  Loads : PMIOPort  Port=2  Side=Right
  connections:
  Gen3 BusLabel/LConn1 -- Bus32/LConn1
  GB28B29T/LConn1 -- B28 to B29/RConn2
  GB26B29F/LConn1 -- B26 to B29/LConn2
  GB7B6F/LConn1 -- B7 to B6/LConn2
  Bus27/RConn1 -- B27 to B26/LConn1
  B26 to B29/RConn1 -- Bus29/LConn1
  GB25B26T/LConn1 -- B25 to B26/RConn2
  B23 to B24/RConn1 -- Bus24/LConn2
  GB23B22T/LConn1 -- B23 to B22/RConn2
  GB18B17T/LConn1 -- B18 to B17/RConn2
  Bus7/RConn1 -- B7 to B6/LConn1
  GB21B22T/LConn1 -- B21 to B22/RConn2
  GB16B24T/LConn1 -- B16 to B24/RConn2
  GB5B4T/LConn1 -- B5 to B4/RConn2
  Bus18/RConn1 -- B18 to B17/LConn1
  Bus15/RConn1 -- B15 to B16/LConn1
  GB19B16T/LConn1 -- B19 to B16/RConn2
  B8 to B7/RConn1 -- Bus7/LConn1
  GB19B16F/LConn1 -- B19 to B16/LConn2
  GB16B17F/LConn1 -- B16 to B17/LConn2
  B14 to B15/RConn1 -- Bus15/LConn1
  Bus21/RConn1 -- B21 to B16/LConn1
  GB39B1T/LConn1 -- B39 to B1/RConn2
  Loads/RConn1 -- LoadBus/RConn1
  B10 to B11/RConn1 -- Bus11/LConn1
  Bus10/RConn1 -- B10 to B11/LConn1
  B13 to B14/RConn1 -- Bus14/LConn2
  GB16B24F/LConn1 -- B16 to B24/LConn2
  GB8B7F/LConn1 -- B8 to B7/LConn2
  Bus8/RConn2 -- B8 to B7/LConn1
  GB9B8T/LConn1 -- B9 to B8/RConn2
  GB13B14F/LConn1 -- B13 to B14/LConn2
  Bus23/RConn2 -- B23 to B24/LConn1
  Bus11/RConn1 -- B11 to B6/LConn1
  GB8B7T/LConn1 -- B8 to B7/RConn2
  GB3B18F/LConn1 -- B3 to B18/LConn2
  B5 to B4/RConn1 -- Bus4/LConn1
  GB11B6T/LConn1 -- B11 to B6/RConn2
  Bus17/RConn1 -- B17 to B27/LConn1
  GB11B6F/LConn1 -- B11 to B6/LConn2
  GB4B3T/LConn1 -- B4 to B3/RConn2
  GB6B5F/LConn1 -- B6 to B5/LConn2
  B39 to B1/RConn1 -- Bus1/LConn1
  GB39B1F/LConn1 -- B39 to B1/LConn2
  B3 to B2/RConn1 -- Bus2/LConn2
  Bus16_1/LConn1 -- B15 to B16/RConn1
  GB2B25T/LConn1 -- B2 to B25/RConn2
  GB7B6T/LConn1 -- B7 to B6/RConn2
  GenBus/LConn7 -- Gen7 GenLabel/LConn1
  B23 to B22/RConn1 -- Bus22/LConn2
  Bus34/RConn1 -- TF B34 to B20/LConn1
  Bus36/LConn1 -- Gen7 BusLabel/LConn1
  GB15B16F/LConn1 -- B15 to B16/LConn2
  Bus18/LConn2 -- Load18 BusLabel/LConn1
  B1 to B2/RConn1 -- Bus2/LConn1
  Bus23/RConn1 -- B23 to B22/LConn1
  LoadBus/LConn15 -- Load27 LoadLabel/LConn1
  LoadBus/LConn18 -- Load31 LoadLabel/LConn1
  Bus32/RConn1 -- TF B32 to B10/LConn1
  GB3B2T/LConn1 -- B3 to B2/RConn2
  LoadBus/LConn14 -- Load26 LoadLabel/LConn1
  LoadBus/LConn16 -- Load28 LoadLabel/LConn1
  LoadBus/LConn12 -- Load24 LoadLabel/LConn1
  TF B2 to B30/RConn1 -- Bus30/LConn1
  Bus26_2/RConn1 -- Load26 BusLabel/LConn1
  B16 to B24/RConn1 -- Bus24/LConn1
  LoadBus/LConn19 -- Load39 LoadLabel/LConn1
  LoadBus/LConn17 -- Load29 LoadLabel/LConn1
  Bus19/RConn1 -- B19 to B16/LConn1
  TF B25 to B37/RConn1 -- Bus37/LConn1
  GB16B17T/LConn1 -- B16 to B17/RConn2
  LoadBus/LConn7 -- Load16 LoadLabel/LConn1
  Bus34/LConn1 -- Gen5 BusLabel/LConn1
  Bus39/LConn2 -- Gen1 BusLabel/LConn1
  Bus3/RConn1 -- B3 to B2/LConn1
  GenBus/LConn2 -- Gen2 GenLabel/LConn1
  LoadBus/LConn11 -- Load23 LoadLabel/LConn1
  LoadBus/LConn10 -- Load21 LoadLabel/LConn1
  Gens/RConn1 -- GenBus/RConn1
  B21 to B16/RConn1 -- Bus16_2/LConn2
  Bus30/RConn1 -- Gen10 BusLabel/LConn1
  LoadBus/LConn2 -- Load4 LoadLabel/LConn1
  Bus16_1/RConn1 -- Fault (Three-Phase)/LConn1 -- B16 to B17/LConn1
  GB23B24F/LConn1 -- B23 to B24/LConn2
  Bus4/LConn2 -- Load4 BusLabel/LConn1
  Bus4/RConn2 -- B4 to B14/LConn1
  GB18B17F/LConn1 -- B18 to B17/LConn2
  B9 to B8/RConn1 -- Bus8/LConn1
  GB26B28F/LConn1 -- B26 to B28/LConn2
  GB4B14T/LConn1 -- B4 to B14/RConn2
  GB10B13T/LConn1 -- B10 to B13/RConn2
  Bus31/LConn2 -- Load31 BusLabel/LConn1
  GB10B11T/LConn1 -- B10 to B11/RConn2
  LoadBus/LConn9 -- Load20 LoadLabel/LConn1
  B19 to B16/RConn1 -- Bus16_1/LConn2 -- Bus16_2/LConn1
  B25 to B26/RConn1 -- Bus26_1/LConn1 -- Bus26_2/LConn1
  LoadBus/LConn6 -- Load15 LoadLabel/LConn1
  Bus8/RConn1 -- B8 to B5/LConn1
  B17 to B27/RConn1 -- Bus27/LConn1
  Bus28/LConn2 -- Load28 BusLabel/LConn1
  Bus9/LConn1 -- B9 to B39/LConn1
  LoadBus/LConn3 -- Load7 LoadLabel/LConn1
  LoadBus/LConn4 -- Load8 LoadLabel/LConn1
  Bus13/RConn1 -- B13 to B14/LConn1
  B4 to B3/RConn1 -- Bus3/LConn1
  Bus3/LConn2 -- Load3 BusLabel/LConn1
  LoadBus/LConn5 -- Load12 LoadLabel/LConn1
  GB23B24T/LConn1 -- B23 to B24/RConn2
  Bus5/RConn1 -- B5 to B4/LConn1
  B2 to B25/RConn1 -- Bus25/LConn1
  Bus23/LConn2 -- Load23 BusLabel/LConn1
  B26 to B28/RConn1 -- Bus28/LConn1
  LoadBus/LConn13 -- Load25 LoadLabel/LConn1
  GB15B16T/LConn1 -- B15 to B16/RConn2
  Bus35/RConn1 -- Gen6 BusLabel/LConn1
  Bus39/RConn1 -- B39 to B1/LConn1
  GB28B29F/LConn1 -- B28 to B29/LConn2
  Bus29/RConn2 -- Load29 BusLabel/LConn1
  GB8B5T/LConn1 -- B8 to B5/RConn2
  Bus25/LConn2 -- Load25 BusLabel/LConn1
  B7 to B6/RConn1 -- Bus6/LConn1
  Bus39/RConn2 -- Load39 BusLabel/LConn1
  GB26B29T/LConn1 -- B26 to B29/RConn2
  Bus27/LConn2 -- Load27 BusLabel/LConn1
  GB8B5F/LConn1 -- B8 to B5/LConn2
  Bus37/RConn1 -- Gen8 BusLabel/LConn1
  GB10B13F/LConn1 -- B10 to B13/LConn2
  GB3B2F/LConn1 -- B3 to B2/LConn2
  GB9B8F/LConn1 -- B9 to B8/LConn2
  GB27B26T/LConn1 -- B27 to B26/RConn2
  LoadBus/LConn1 -- Load3 LoadLabel/LConn1
  GenBus/LConn6 -- Gen6 GenLabel/LConn1
  B21 to B22/RConn1 -- Bus22/LConn1
  GB14B15F/LConn1 -- B14 to B15/LConn2
  GB17B27T/LConn1 -- B17 to B27/RConn2
  Bus9/RConn1 -- B9 to B8/LConn1
  B3 to B18/RConn1 -- Bus18/LConn1
  Bus16_1/RConn2 -- B16 to B24/LConn1
  GB25B26F/LConn1 -- B25 to B26/LConn2
  GenBus/LConn9 -- Gen9 GenLabel/LConn1
  GB21B16T/LConn1 -- B21 to B16/RConn2
  Bus7/LConn2 -- Load7 BusLabel/LConn1
  Bus33/LConn1 -- Gen4 BusLabel/LConn1
  Bus31/RConn1 -- TF B31 to B6/LConn1
  GB13B14T/LConn1 -- B13 to B14/RConn2
  GenBus/LConn8 -- Gen8 GenLabel/LConn1
  GB4B14F/LConn1 -- B4 to B14/LConn2
  GB26B28T/LConn1 -- B26 to B28/RConn2
  Bus1/RConn1 -- B1 to B2/LConn1
  GenBus/LConn5 -- Gen5 GenLabel/LConn1
  GB4B3F/LConn1 -- B4 to B3/LConn2
  Bus33/RConn1 -- TF B33 to B19/LConn1
  GB21B16F/LConn1 -- B21 to B16/LConn2
  GB1B2F/LConn1 -- B1 to B2/LConn2
  Bus8/LConn2 -- Load8 BusLabel/LConn1
  GB10B11F/LConn1 -- B10 to B11/LConn2
  Bus26_1/RConn1 -- B26 to B28/LConn1
  Bus28/RConn1 -- B28 to B29/LConn1
  TF B38 to B29/RConn1 -- Bus29/RConn1
  GB2B25F/LConn1 -- B2 to B25/LConn2
  GenBus/LConn1 -- Gen10 GenLabel/LConn1
  GenBus/LConn4 -- Gen4 GenLabel/LConn1
  LoadBus/LConn8 -- Load18 LoadLabel/LConn1
  Bus12/RConn1 -- Load12 BusLabel/LConn1
  GB23B22F/LConn1 -- B23 to B22/LConn2
  Gen1 GenLabel/LConn1 -- Solver Configuration/RConn1 -- GenBus/LConn10
  Bus36/RConn1 -- TF B36 to B23/LConn1
  TF B36 to B23/RConn1 -- Bus23/LConn1
  Bus3/RConn2 -- B3 to B18/LConn1
  TF B22 to B35/RConn1 -- Bus35/LConn1
  GB5B4F/LConn1 -- B5 to B4/LConn2
  GB9B39T/LConn1 -- B9 to B39/RConn2
  GB9B39F/LConn1 -- B9 to B39/LConn2
  Bus24/RConn1 -- Load24 BusLabel/LConn1
  TF B20 to B19/RConn1 -- Bus19/LConn1
  B28 to B29/RConn1 -- Bus29/LConn2
  TF B13 to B12/RConn1 -- Bus12/LConn2
  Bus14/RConn1 -- B14 to B15/LConn1
  Bus11/LConn2 -- TF B11 to B12/LConn1
  Bus16_2/RConn1 -- Load16 BusLabel/LConn1
  GB14B15T/LConn1 -- B14 to B15/RConn2
  GB6B5T/LConn1 -- B6 to B5/RConn2
  GB27B26F/LConn1 -- B27 to B26/LConn2
  GB1B2T/LConn1 -- B1 to B2/RConn2
  GB3B18T/LConn1 -- B3 to B18/RConn2
  GenBus/LConn3 -- Gen3 GenLabel/LConn1
  Bus20/RConn1 -- TF B20 to B19/LConn1
  TF B34 to B20/RConn1 -- Bus20/LConn1
  Bus4/RConn1 -- B4 to B3/LConn1
  TF B11 to B12/RConn1 -- Bus12/LConn1
  Bus38/LConn1 -- Gen9 BusLabel/LConn1
  Bus20/LConn2 -- Load20 BusLabel/LConn1
  Bus26_1/RConn2 -- B26 to B29/LConn1
  Bus38/RConn1 -- TF B38 to B29/LConn1
  GB17B27F/LConn1 -- B17 to B27/LConn2
  B9 to B39/RConn1 -- Bus39/LConn1
  Bus15/LConn2 -- Load15 BusLabel/LConn1
  GB21B22F/LConn1 -- B21 to B22/LConn2
  B4 to B14/RConn1 -- Bus14/LConn1
  B27 to B26/RConn1 -- Bus26_1/LConn2
  Bus6/RConn1 -- B6 to B5/LConn1
  Bus22/RConn1 -- TF B22 to B35/LConn1
  Bus31/LConn1 -- Gen2 BusLabel/LConn1
  TF B33 to B19/RConn1 -- Bus19/LConn2
  TF B31 to B6/RConn1 -- Bus6/LConn2
  B11 to B6/RConn1 -- Bus6/RConn2
  B21 to B22/LConn1 -- Bus21/LConn2
  Load21 BusLabel/LConn1 -- Bus21/LConn1
  Bus25/RConn2 -- B25 to B26/LConn1
  Bus25/RConn1 -- TF B25 to B37/LConn1
  B2 to B25/LConn1 -- Bus2/RConn2
  TF B2 to B30/LConn1 -- Bus2/RConn1
  B8 to B5/RConn1 -- Bus5/LConn1
  B6 to B5/RConn1 -- Bus5/LConn2
  B10 to B13/RConn1 -- Bus13/LConn2
  TF B13 to B12/LConn1 -- Bus13/LConn1
  Bus10/LConn1 -- TF B32 to B10/RConn1
  B10 to B13/LConn1 -- Bus10/LConn2
  B16 to B17/RConn1 -- Bus17/LConn2
  B18 to B17/RConn1 -- Bus17/LConn1
